simulink model "ANNModel"  (R2020a)
settings: Solver=VariableStepAuto  StartTime=0.0  StopTime=10.0  RelTol=1e-3
values from neighbouring files (symbols this model uses):
  dijastolniPritisak = str2num(get(handles.edit2,'string'))    [GUI.m]
  glukoza = str2num(get(handles.edit4,'string'))    [GUI.m]
  obimStruka = str2num(get(handles.edit1,'string'))    [GUI.m]
  sistolniPritisak = str2num(get(handles.edit3,'string'))    [GUI.m]
  trigliceridi = str2num(get(handles.edit5,'string'))    [GUI.m]
undefined symbols (not defined in the file or in its folder): hdlCartesian2PolarSetting
libraries: neural x255
(part 2 of 4)

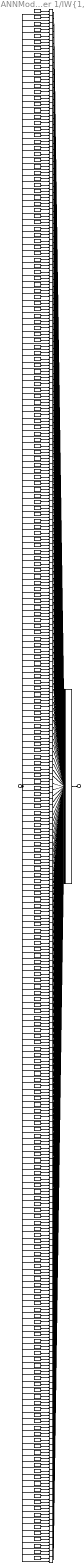
== system ANNModel/Function Fitting Neural Network/Layer 1/IW{1,1} ==
  "pd{1,1}" : Inport  PortDimensions=6
      mask Display: e = 0.06;c1 = [120 230 180]/255;c2 = ([120 230 180]+0)/(256+128);c3 = ([120 230 180]+128)/(256+128);patch([0 1 1 0],[0 0 1 1],c1);patch([0 1 1 1-e 1-e 0+e],[0 0 1 1-e 0+e 0+e],c2);patch([0 0 1 1-e 0+e 0+e],[0 1 1 1-e 1-e 0+e],c3);plot([0 1 1 0 0],[0 0 1 1 0]);
  "IW{1,1}(1,:)'" : Constant  Value=[0.287796190022346631831595686890068463981151580810546875;-1.9089648936896697062337580064195208251476287841796875;2.23832582693165793585876599536277353763580322265625;-1.4430056380304934204872324698953889310359954833984375;1.1609374416815703145999805201427079737186431884765625;-0.89544104034703086991697773555642925202846527099609375]
      mask Display: e = 0.06;c1 = [120 150 230]/255;c2 = ([120 150 230]+0)/383;c3 = ([120 150 230]+128)/383;patch([0 1 1 0],[0 0 1 1],c1);patch([0 1 1 1-e 1-e 0+e],[0 0 1 1-e 0+e 0+e],c2);patch([0 0 1 1-e 0+e 0+e],[0 1 1 1-e 1-e 0+e],c3);plot([0 1 1 0 0],[0 0 1 1 0]);disp('Weights');
  "IW{1,1}(10,:)'" : Constant  Value=[1.171278222760385734346755270962603390216827392578125;2.23653260652877516889702746993862092494964599609375;-0.01489189259019494011859752191639927332289516925811767578125;1.1450374400558178678011245210655033588409423828125;-1.8858407208954393041722141788341104984283447265625;-1.1545086890824993730575442896224558353424072265625]
      mask Display: e = 0.06;c1 = [120 150 230]/255;c2 = ([120 150 230]+0)/383;c3 = ([120 150 230]+128)/383;patch([0 1 1 0],[0 0 1 1],c1);patch([0 1 1 1-e 1-e 0+e],[0 0 1 1-e 0+e 0+e],c2);patch([0 0 1 1-e 0+e 0+e],[0 1 1 1-e 1-e 0+e],c3);plot([0 1 1 0 0],[0 0 1 1 0]);disp('Weights');
  "IW{1,1}(100,:)'" : Constant  Value=[1.663125101440811715036716122995130717754364013671875;-1.3324885457119133302938962515327148139476776123046875;1.40799126740946167757329021696932613849639892578125;-0.82146034869195483363313314839615486562252044677734375;-1.30446631893276876468235059292055666446685791015625;1.865641928271901672786725612240843474864959716796875]
      mask Display: e = 0.06;c1 = [120 150 230]/255;c2 = ([120 150 230]+0)/383;c3 = ([120 150 230]+128)/383;patch([0 1 1 0],[0 0 1 1],c1);patch([0 1 1 1-e 1-e 0+e],[0 0 1 1-e 0+e 0+e],c2);patch([0 0 1 1-e 0+e 0+e],[0 1 1 1-e 1-e 0+e],c3);plot([0 1 1 0 0],[0 0 1 1 0]);disp('Weights');
  "IW{1,1}(101,:)'" : Constant  Value=[1.0994399106034584701063749889726750552654266357421875;-1.94404946470914552492104121483862400054931640625;1.677632189897698022917893467820249497890472412109375;0.94695867514827247735098580960766412317752838134765625;-1.9872291711378233802776094307773746550083160400390625;0.461357489766259398766834465277497656643390655517578125]
      mask Display: e = 0.06;c1 = [120 150 230]/255;c2 = ([120 150 230]+0)/383;c3 = ([120 150 230]+128)/383;patch([0 1 1 0],[0 0 1 1],c1);patch([0 1 1 1-e 1-e 0+e],[0 0 1 1-e 0+e 0+e],c2);patch([0 0 1 1-e 0+e 0+e],[0 1 1 1-e 1-e 0+e],c3);plot([0 1 1 0 0],[0 0 1 1 0]);disp('Weights');
  "IW{1,1}(102,:)'" : Constant  Value=[-1.7449163202875137557157358969561755657196044921875;-0.9713941744906346986709877455723471939563751220703125;0.64768518707501609998899994025123305618762969970703125;1.7546407768395833048913345919572748243808746337890625;-2.00079378864895662815115429111756384372711181640625;-0.89837385215088028100893779992475174367427825927734375]
      mask Display: e = 0.06;c1 = [120 150 230]/255;c2 = ([120 150 230]+0)/383;c3 = ([120 150 230]+128)/383;patch([0 1 1 0],[0 0 1 1],c1);patch([0 1 1 1-e 1-e 0+e],[0 0 1 1-e 0+e 0+e],c2);patch([0 0 1 1-e 0+e 0+e],[0 1 1 1-e 1-e 0+e],c3);plot([0 1 1 0 0],[0 0 1 1 0]);disp('Weights');
  "IW{1,1}(103,:)'" : Constant  Value=[-1.8700045070212301112633213051594793796539306640625;1.1538376759129302939754779799841344356536865234375;1.3190542580864479393909505233750678598880767822265625;0.03391908880042536489352045236955746077001094818115234375;-1.42011272119921638790174256428144872188568115234375;-1.93961983755487921143867424689233303070068359375]
      mask Display: e = 0.06;c1 = [120 150 230]/255;c2 = ([120 150 230]+0)/383;c3 = ([120 150 230]+128)/383;patch([0 1 1 0],[0 0 1 1],c1);patch([0 1 1 1-e 1-e 0+e],[0 0 1 1-e 0+e 0+e],c2);patch([0 0 1 1-e 0+e 0+e],[0 1 1 1-e 1-e 0+e],c3);plot([0 1 1 0 0],[0 0 1 1 0]);disp('Weights');
  "IW{1,1}(104,:)'" : Constant  Value=[-1.9055149673777507235428174681146629154682159423828125;1.7368910868478895093147684747236780822277069091796875;-1.3775290622561680020652374878409318625926971435546875;-1.358849834002237688679315397166647017002105712890625;0.60619469881785248421834921828121878206729888916015625;-0.9743336437083087719912555257906205952167510986328125]
      mask Display: e = 0.06;c1 = [120 150 230]/255;c2 = ([120 150 230]+0)/383;c3 = ([120 150 230]+128)/383;patch([0 1 1 0],[0 0 1 1],c1);patch([0 1 1 1-e 1-e 0+e],[0 0 1 1-e 0+e 0+e],c2);patch([0 0 1 1-e 0+e 0+e],[0 1 1 1-e 1-e 0+e],c3);plot([0 1 1 0 0],[0 0 1 1 0]);disp('Weights');
  "IW{1,1}(105,:)'" : Constant  Value=[-1.2927935449414416080315959334257058799266815185546875;-2.876361513359648736098961308016441762447357177734375;0.144244721152042953971061933771125040948390960693359375;0.25663209727781233215893053056788630783557891845703125;0.58464584217745552141565212878049351274967193603515625;1.4202487725735595258669263785122893750667572021484375]
      mask Display: e = 0.06;c1 = [120 150 230]/255;c2 = ([120 150 230]+0)/383;c3 = ([120 150 230]+128)/383;patch([0 1 1 0],[0 0 1 1],c1);patch([0 1 1 1-e 1-e 0+e],[0 0 1 1-e 0+e 0+e],c2);patch([0 0 1 1-e 0+e 0+e],[0 1 1 1-e 1-e 0+e],c3);plot([0 1 1 0 0],[0 0 1 1 0]);disp('Weights');
  "IW{1,1}(106,:)'" : Constant  Value=[1.3715068673942329979809073847718536853790283203125;-1.8144972173688571626115617618779651820659637451171875;-1.659935553705334410068417128059081733226776123046875;-0.85473222772530255131329113282845355570316314697265625;1.8349805103916019266563353085075505077838897705078125;0.38149494665385663694223694619722664356231689453125]
      mask Display: e = 0.06;c1 = [120 150 230]/255;c2 = ([120 150 230]+0)/383;c3 = ([120 150 230]+128)/383;patch([0 1 1 0],[0 0 1 1],c1);patch([0 1 1 1-e 1-e 0+e],[0 0 1 1-e 0+e 0+e],c2);patch([0 0 1 1-e 0+e 0+e],[0 1 1 1-e 1-e 0+e],c3);plot([0 1 1 0 0],[0 0 1 1 0]);disp('Weights');
  "IW{1,1}(107,:)'" : Constant  Value=[-2.393727032684455746647245177882723510265350341796875;1.20553523596906675408035880536772310733795166015625;1.9170047359852304680316592566668987274169921875;-0.74935458790647413440666468886774964630603790283203125;0.827817899649488708746503107249736785888671875;0.400360585595414264492575284748454578220844268798828125]
      mask Display: e = 0.06;c1 = [120 150 230]/255;c2 = ([120 150 230]+0)/383;c3 = ([120 150 230]+128)/383;patch([0 1 1 0],[0 0 1 1],c1);patch([0 1 1 1-e 1-e 0+e],[0 0 1 1-e 0+e 0+e],c2);patch([0 0 1 1-e 0+e 0+e],[0 1 1 1-e 1-e 0+e],c3);plot([0 1 1 0 0],[0 0 1 1 0]);disp('Weights');
  "IW{1,1}(108,:)'" : Constant  Value=[0.58456128724172040644901926498278044164180755615234375;0.451576994767699135824301492903032340109348297119140625;-1.1295822098068881711441235893289558589458465576171875;-2.064741374551308350504541522241197526454925537109375;-0.330601885825315855438333301208331249654293060302734375;2.430200037822459080416592769324779510498046875]
      mask Display: e = 0.06;c1 = [120 150 230]/255;c2 = ([120 150 230]+0)/383;c3 = ([120 150 230]+128)/383;patch([0 1 1 0],[0 0 1 1],c1);patch([0 1 1 1-e 1-e 0+e],[0 0 1 1-e 0+e 0+e],c2);patch([0 0 1 1-e 0+e 0+e],[0 1 1 1-e 1-e 0+e],c3);plot([0 1 1 0 0],[0 0 1 1 0]);disp('Weights');
  "IW{1,1}(109,:)'" : Constant  Value=[2.180394306035542850707997786230407655239105224609375;-1.1778737761314694854064555329387076199054718017578125;2.11431337255463613900019481661729514598846435546875;1.1326449641214388908139198974822647869586944580078125;-0.67526687425978793033465308326412923634052276611328125;-0.07736857178589713612826272992606391198933124542236328125]
      mask Display: e = 0.06;c1 = [120 150 230]/255;c2 = ([120 150 230]+0)/383;c3 = ([120 150 230]+128)/383;patch([0 1 1 0],[0 0 1 1],c1);patch([0 1 1 1-e 1-e 0+e],[0 0 1 1-e 0+e 0+e],c2);patch([0 0 1 1-e 0+e 0+e],[0 1 1 1-e 1-e 0+e],c3);plot([0 1 1 0 0],[0 0 1 1 0]);disp('Weights');
  "IW{1,1}(11,:)'" : Constant  Value=[1.6315197961081737698663118862896226346492767333984375;-0.2131235197336888431696166890105814673006534576416015625;-0.815333650431852685613876019488088786602020263671875;2.37567903756769993606212665326893329620361328125;0.2414189732595966031425405162735842168331146240234375;-1.881982712422992864986781569314189255237579345703125]
      mask Display: e = 0.06;c1 = [120 150 230]/255;c2 = ([120 150 230]+0)/383;c3 = ([120 150 230]+128)/383;patch([0 1 1 0],[0 0 1 1],c1);patch([0 1 1 1-e 1-e 0+e],[0 0 1 1-e 0+e 0+e],c2);patch([0 0 1 1-e 0+e 0+e],[0 1 1 1-e 1-e 0+e],c3);plot([0 1 1 0 0],[0 0 1 1 0]);disp('Weights');
  "IW{1,1}(110,:)'" : Constant  Value=[1.871977750312087795947491031256504356861114501953125;1.9065529752603100899221999497967772185802459716796875;1.10235750480877481294328390504233539104461669921875;-0.12466250876593264196312560443402617238461971282958984375;-1.852760848460142550919727000291459262371063232421875;-0.83235765970877928499049858146463520824909210205078125]
      mask Display: e = 0.06;c1 = [120 150 230]/255;c2 = ([120 150 230]+0)/383;c3 = ([120 150 230]+128)/383;patch([0 1 1 0],[0 0 1 1],c1);patch([0 1 1 1-e 1-e 0+e],[0 0 1 1-e 0+e 0+e],c2);patch([0 0 1 1-e 0+e 0+e],[0 1 1 1-e 1-e 0+e],c3);plot([0 1 1 0 0],[0 0 1 1 0]);disp('Weights');
  "IW{1,1}(111,:)'" : Constant  Value=[2.715895301511082937651053725858218967914581298828125;-0.1845621160394123327908033616040484048426151275634765625;-1.1417582632765548300568525519338436424732208251953125;0.1105548504869580117571103983209468424320220947265625;-1.873172352911395943664274454931728541851043701171875;0.227437856943576932611250640547950752079486846923828125]
      mask Display: e = 0.06;c1 = [120 150 230]/255;c2 = ([120 150 230]+0)/383;c3 = ([120 150 230]+128)/383;patch([0 1 1 0],[0 0 1 1],c1);patch([0 1 1 1-e 1-e 0+e],[0 0 1 1-e 0+e 0+e],c2);patch([0 0 1 1-e 0+e 0+e],[0 1 1 1-e 1-e 0+e],c3);plot([0 1 1 0 0],[0 0 1 1 0]);disp('Weights');
  "IW{1,1}(112,:)'" : Constant  Value=[-2.865597023084187622288254715385846793651580810546875;0.55121427735391181901292156908311881124973297119140625;-1.3240199081592951557695414521731436252593994140625;1.03647974126135533623482842813245952129364013671875;-0.05899074146290349263122010370352654717862606048583984375;0.8046617095188033363939439368550665676593780517578125]
      mask Display: e = 0.06;c1 = [120 150 230]/255;c2 = ([120 150 230]+0)/383;c3 = ([120 150 230]+128)/383;patch([0 1 1 0],[0 0 1 1],c1);patch([0 1 1 1-e 1-e 0+e],[0 0 1 1-e 0+e 0+e],c2);patch([0 0 1 1-e 0+e 0+e],[0 1 1 1-e 1-e 0+e],c3);plot([0 1 1 0 0],[0 0 1 1 0]);disp('Weights');
  "IW{1,1}(113,:)'" : Constant  Value=[-0.310917571005290327423864482625504024326801300048828125;-0.785412215734894392227261050720699131488800048828125;-0.74616182881038906060666704433970153331756591796875;-2.010551802483051542225211960612796247005462646484375;-0.78039983614209218476531759733916260302066802978515625;-2.38104318153131000457278787507675588130950927734375]
      mask Display: e = 0.06;c1 = [120 150 230]/255;c2 = ([120 150 230]+0)/383;c3 = ([120 150 230]+128)/383;patch([0 1 1 0],[0 0 1 1],c1);patch([0 1 1 1-e 1-e 0+e],[0 0 1 1-e 0+e 0+e],c2);patch([0 0 1 1-e 0+e 0+e],[0 1 1 1-e 1-e 0+e],c3);plot([0 1 1 0 0],[0 0 1 1 0]);disp('Weights');
  "IW{1,1}(114,:)'" : Constant  Value=[-0.74016223365661082400634995792643167078495025634765625;-1.5122705125749271726220968048437498509883880615234375;-0.1761518912334952557952050256062648259103298187255859375;1.880329117756179169163033293443731963634490966796875;-1.4859694564245569115001899263006635010242462158203125;-1.9323614898229741765334210867877118289470672607421875]
      mask Display: e = 0.06;c1 = [120 150 230]/255;c2 = ([120 150 230]+0)/383;c3 = ([120 150 230]+128)/383;patch([0 1 1 0],[0 0 1 1],c1);patch([0 1 1 1-e 1-e 0+e],[0 0 1 1-e 0+e 0+e],c2);patch([0 0 1 1-e 0+e 0+e],[0 1 1 1-e 1-e 0+e],c3);plot([0 1 1 0 0],[0 0 1 1 0]);disp('Weights');
  "IW{1,1}(115,:)'" : Constant  Value=[-0.026530589428871730051096022862111567519605159759521484375;1.791368487953234112097788965911604464054107666015625;-0.038144839645352486556806326234436710365116596221923828125;1.3401104395405099012350547127425670623779296875;-1.646448745847335803915711949230171740055084228515625;-2.112684036522342267971907858736813068389892578125]
      mask Display: e = 0.06;c1 = [120 150 230]/255;c2 = ([120 150 230]+0)/383;c3 = ([120 150 230]+128)/383;patch([0 1 1 0],[0 0 1 1],c1);patch([0 1 1 1-e 1-e 0+e],[0 0 1 1-e 0+e 0+e],c2);patch([0 0 1 1-e 0+e 0+e],[0 1 1 1-e 1-e 0+e],c3);plot([0 1 1 0 0],[0 0 1 1 0]);disp('Weights');
  "IW{1,1}(116,:)'" : Constant  Value=[1.5812661283949827062400572685874067246913909912109375;1.767995003883346072370841284282505512237548828125;-0.346389538115326522937920117328758351504802703857421875;0.431948010021581618733677032651030458509922027587890625;-1.8555401924967716009717833003378473222255706787109375;-1.704494922192528516546872197068296372890472412109375]
      mask Display: e = 0.06;c1 = [120 150 230]/255;c2 = ([120 150 230]+0)/383;c3 = ([120 150 230]+128)/383;patch([0 1 1 0],[0 0 1 1],c1);patch([0 1 1 1-e 1-e 0+e],[0 0 1 1-e 0+e 0+e],c2);patch([0 0 1 1-e 0+e 0+e],[0 1 1 1-e 1-e 0+e],c3);plot([0 1 1 0 0],[0 0 1 1 0]);disp('Weights');
  "IW{1,1}(117,:)'" : Constant  Value=[-1.2368412784026714401619528871378861367702484130859375;2.249261562349092802293171189376153051853179931640625;0.69995883312456508296151014292263425886631011962890625;0.089521939729461597057280641820398159325122833251953125;1.177139767436751416340712239616550505161285400390625;-1.871593531701182921977988371509127318859100341796875]
      mask Display: e = 0.06;c1 = [120 150 230]/255;c2 = ([120 150 230]+0)/383;c3 = ([120 150 230]+128)/383;patch([0 1 1 0],[0 0 1 1],c1);patch([0 1 1 1-e 1-e 0+e],[0 0 1 1-e 0+e 0+e],c2);patch([0 0 1 1-e 0+e 0+e],[0 1 1 1-e 1-e 0+e],c3);plot([0 1 1 0 0],[0 0 1 1 0]);disp('Weights');
  "IW{1,1}(118,:)'" : Constant  Value=[0.60304962449617349751207484587212093174457550048828125;-1.124505931275801007274139919900335371494293212890625;-2.198952551738090566146865967311896383762359619140625;-1.0802931006421128135031040073954500257968902587890625;-0.89556215647179382433051841871929354965686798095703125;1.944692625398790841728668965515680611133575439453125]
      mask Display: e = 0.06;c1 = [120 150 230]/255;c2 = ([120 150 230]+0)/383;c3 = ([120 150 230]+128)/383;patch([0 1 1 0],[0 0 1 1],c1);patch([0 1 1 1-e 1-e 0+e],[0 0 1 1-e 0+e 0+e],c2);patch([0 0 1 1-e 0+e 0+e],[0 1 1 1-e 1-e 0+e],c3);plot([0 1 1 0 0],[0 0 1 1 0]);disp('Weights');
  "IW{1,1}(119,:)'" : Constant  Value=[1.482736380110039942081812114338390529155731201171875;-0.6897419204355188515620511680026538670063018798828125;-0.7221616959874612717840136610902845859527587890625;1.878595439276721013044380015344358980655670166015625;1.0859477348788020290015765567659400403499603271484375;-2.0840921036468404992092473548837006092071533203125]
      mask Display: e = 0.06;c1 = [120 150 230]/255;c2 = ([120 150 230]+0)/383;c3 = ([120 150 230]+128)/383;patch([0 1 1 0],[0 0 1 1],c1);patch([0 1 1 1-e 1-e 0+e],[0 0 1 1-e 0+e 0+e],c2);patch([0 0 1 1-e 0+e 0+e],[0 1 1 1-e 1-e 0+e],c3);plot([0 1 1 0 0],[0 0 1 1 0]);disp('Weights');
  "IW{1,1}(12,:)'" : Constant  Value=[1.5455546652351539460568119466188363730907440185546875;-1.5484718191601032355464440115611068904399871826171875;1.7087711909293610279547692698542959988117218017578125;1.785864571327177241499839510652236640453338623046875;1.4157761391038483633764144542510621249675750732421875;-1.5651679421094624178323329033446498215198516845703125]
      mask Display: e = 0.06;c1 = [120 150 230]/255;c2 = ([120 150 230]+0)/383;c3 = ([120 150 230]+128)/383;patch([0 1 1 0],[0 0 1 1],c1);patch([0 1 1 1-e 1-e 0+e],[0 0 1 1-e 0+e 0+e],c2);patch([0 0 1 1-e 0+e 0+e],[0 1 1 1-e 1-e 0+e],c3);plot([0 1 1 0 0],[0 0 1 1 0]);disp('Weights');
  "IW{1,1}(120,:)'" : Constant  Value=[1.288138171530183395674384883022867143154144287109375;1.7591734283443953845704754712642170488834381103515625;-2.546961424497379056219870108179748058319091796875;0.26152048374034009281530188673059456050395965576171875;-0.75234596311726098516459160236991010606288909912109375;-0.396041123684448159725235427686129696667194366455078125]
      mask Display: e = 0.06;c1 = [120 150 230]/255;c2 = ([120 150 230]+0)/383;c3 = ([120 150 230]+128)/383;patch([0 1 1 0],[0 0 1 1],c1);patch([0 1 1 1-e 1-e 0+e],[0 0 1 1-e 0+e 0+e],c2);patch([0 0 1 1-e 0+e 0+e],[0 1 1 1-e 1-e 0+e],c3);plot([0 1 1 0 0],[0 0 1 1 0]);disp('Weights');
  "IW{1,1}(121,:)'" : Constant  Value=[1.6789379176582592823052664243732579052448272705078125;-2.06756931519347464387692525633610785007476806640625;-0.83431558709326869571754059506929479539394378662109375;-0.11764986868161116106978880679889698512852191925048828125;-0.741921904057246894836907813441939651966094970703125;1.7037612455942536815456378462840802967548370361328125]
      mask Display: e = 0.06;c1 = [120 150 230]/255;c2 = ([120 150 230]+0)/383;c3 = ([120 150 230]+128)/383;patch([0 1 1 0],[0 0 1 1],c1);patch([0 1 1 1-e 1-e 0+e],[0 0 1 1-e 0+e 0+e],c2);patch([0 0 1 1-e 0+e 0+e],[0 1 1 1-e 1-e 0+e],c3);plot([0 1 1 0 0],[0 0 1 1 0]);disp('Weights');
  "IW{1,1}(122,:)'" : Constant  Value=[-2.597069193765010997054787367233075201511383056640625;0.443010847045192390769585699672461487352848052978515625;-0.916897332638182849251506922882981598377227783203125;1.6149206099324933116889724260545335710048675537109375;-1.4291647808392660135012874889071099460124969482421875;-0.011755427704555405921116317813357454724609851837158203125]
      mask Display: e = 0.06;c1 = [120 150 230]/255;c2 = ([120 150 230]+0)/383;c3 = ([120 150 230]+128)/383;patch([0 1 1 0],[0 0 1 1],c1);patch([0 1 1 1-e 1-e 0+e],[0 0 1 1-e 0+e 0+e],c2);patch([0 0 1 1-e 0+e 0+e],[0 1 1 1-e 1-e 0+e],c3);plot([0 1 1 0 0],[0 0 1 1 0]);disp('Weights');
  "IW{1,1}(123,:)'" : Constant  Value=[1.82950962756301027667404923704452812671661376953125;-0.766808582879284994504587302799336612224578857421875;-1.96057973625015602436860717716626822948455810546875;1.0438555136353444563468428896158002316951751708984375;-0.937696667328782762496075520175509154796600341796875;-1.5015461343558171858347805027733556926250457763671875]
      mask Display: e = 0.06;c1 = [120 150 230]/255;c2 = ([120 150 230]+0)/383;c3 = ([120 150 230]+128)/383;patch([0 1 1 0],[0 0 1 1],c1);patch([0 1 1 1-e 1-e 0+e],[0 0 1 1-e 0+e 0+e],c2);patch([0 0 1 1-e 0+e 0+e],[0 1 1 1-e 1-e 0+e],c3);plot([0 1 1 0 0],[0 0 1 1 0]);disp('Weights');
  "IW{1,1}(124,:)'" : Constant  Value=[-1.717308648500118994917329473537392914295196533203125;-0.1143933240111000559924292474534013308584690093994140625;0.70796833666341374424746391014195978641510009765625;1.6833517489322911142579641818883828818798065185546875;-1.6455079596563706445522257126867771148681640625;1.8053204278844316998942076679668389260768890380859375]
      mask Display: e = 0.06;c1 = [120 150 230]/255;c2 = ([120 150 230]+0)/383;c3 = ([120 150 230]+128)/383;patch([0 1 1 0],[0 0 1 1],c1);patch([0 1 1 1-e 1-e 0+e],[0 0 1 1-e 0+e 0+e],c2);patch([0 0 1 1-e 0+e 0+e],[0 1 1 1-e 1-e 0+e],c3);plot([0 1 1 0 0],[0 0 1 1 0]);disp('Weights');
  "IW{1,1}(125,:)'" : Constant  Value=[1.2768026276094157633878012347850017249584197998046875;-1.4743738311023104614605472306720912456512451171875;0.689266690328770526008383967564441263675689697265625;0.449442201861272982998940506149665452539920806884765625;1.553334665702312822332942232606001198291778564453125;2.238972463563259740482180859544314444065093994140625]
      mask Display: e = 0.06;c1 = [120 150 230]/255;c2 = ([120 150 230]+0)/383;c3 = ([120 150 230]+128)/383;patch([0 1 1 0],[0 0 1 1],c1);patch([0 1 1 1-e 1-e 0+e],[0 0 1 1-e 0+e 0+e],c2);patch([0 0 1 1-e 0+e 0+e],[0 1 1 1-e 1-e 0+e],c3);plot([0 1 1 0 0],[0 0 1 1 0]);disp('Weights');
  "IW{1,1}(126,:)'" : Constant  Value=[1.185869669339465470869754426530562341213226318359375;-1.8183989232825459314568661284283734858036041259765625;1.4622955843601552761157336135511286556720733642578125;-1.31858677302676507991918697371147572994232177734375;-1.3866742775623348560287695363513194024562835693359375;0.8449734256742991167499212679103948175907135009765625]
      mask Display: e = 0.06;c1 = [120 150 230]/255;c2 = ([120 150 230]+0)/383;c3 = ([120 150 230]+128)/383;patch([0 1 1 0],[0 0 1 1],c1);patch([0 1 1 1-e 1-e 0+e],[0 0 1 1-e 0+e 0+e],c2);patch([0 0 1 1-e 0+e 0+e],[0 1 1 1-e 1-e 0+e],c3);plot([0 1 1 0 0],[0 0 1 1 0]);disp('Weights');
  "IW{1,1}(127,:)'" : Constant  Value=[-1.5208700661502623230347808203077875077724456787109375;0.36918303584951883689058149684569798409938812255859375;-0.67113679415553428864171792156412266194820404052734375;-1.609631995417881711318841553293168544769287109375;-1.9015268710997628165415562762063927948474884033203125;-1.85020841591162987782581694773398339748382568359375]
      mask Display: e = 0.06;c1 = [120 150 230]/255;c2 = ([120 150 230]+0)/383;c3 = ([120 150 230]+128)/383;patch([0 1 1 0],[0 0 1 1],c1);patch([0 1 1 1-e 1-e 0+e],[0 0 1 1-e 0+e 0+e],c2);patch([0 0 1 1-e 0+e 0+e],[0 1 1 1-e 1-e 0+e],c3);plot([0 1 1 0 0],[0 0 1 1 0]);disp('Weights');
  "IW{1,1}(128,:)'" : Constant  Value=[2.244153766149360240689247802947647869586944580078125;-0.285950788072386996585549923111102543771266937255859375;0.75772497186099785349000512724160216748714447021484375;-1.8382734286454243122221896555856801569461822509765625;-1.05364333862193060298295677057467401027679443359375;-1.5863157094262325674804969821707345545291900634765625]
      mask Display: e = 0.06;c1 = [120 150 230]/255;c2 = ([120 150 230]+0)/383;c3 = ([120 150 230]+128)/383;patch([0 1 1 0],[0 0 1 1],c1);patch([0 1 1 1-e 1-e 0+e],[0 0 1 1-e 0+e 0+e],c2);patch([0 0 1 1-e 0+e 0+e],[0 1 1 1-e 1-e 0+e],c3);plot([0 1 1 0 0],[0 0 1 1 0]);disp('Weights');
  "IW{1,1}(129,:)'" : Constant  Value=[-1.3295196024708582083206920287921093404293060302734375;-0.98565154486492290164534324503620155155658721923828125;0.60676632133203156627132557332515716552734375;-1.672370422375341281195915144053287804126739501953125;1.6587910150941505005306453313096426427364349365234375;-1.8893294430765006364225655488553456962108612060546875]
      mask Display: e = 0.06;c1 = [120 150 230]/255;c2 = ([120 150 230]+0)/383;c3 = ([120 150 230]+128)/383;patch([0 1 1 0],[0 0 1 1],c1);patch([0 1 1 1-e 1-e 0+e],[0 0 1 1-e 0+e 0+e],c2);patch([0 0 1 1-e 0+e 0+e],[0 1 1 1-e 1-e 0+e],c3);plot([0 1 1 0 0],[0 0 1 1 0]);disp('Weights');
  "IW{1,1}(13,:)'" : Constant  Value=[0.81921892677472640809099857506225816905498504638671875;1.568457929113170390422737909830175340175628662109375;2.04499941443174382271763533935882151126861572265625;-1.5514905638126545994737170985899865627288818359375;-1.529102764073087872276346388389356434345245361328125;-0.92744381079182913740766025512129999697208404541015625]
      mask Display: e = 0.06;c1 = [120 150 230]/255;c2 = ([120 150 230]+0)/383;c3 = ([120 150 230]+128)/383;patch([0 1 1 0],[0 0 1 1],c1);patch([0 1 1 1-e 1-e 0+e],[0 0 1 1-e 0+e 0+e],c2);patch([0 0 1 1-e 0+e 0+e],[0 1 1 1-e 1-e 0+e],c3);plot([0 1 1 0 0],[0 0 1 1 0]);disp('Weights');
  "IW{1,1}(130,:)'" : Constant  Value=[2.408864728766730411990693028201349079608917236328125;-0.423623329771535550580807694132090546190738677978515625;-1.1495083404988843955862876100582070648670196533203125;-0.58093209613445784267327098859823308885097503662109375;-2.0011779217500862415590745513327419757843017578125;-0.2364424998863863536247009733415325172245502471923828125]
      mask Display: e = 0.06;c1 = [120 150 230]/255;c2 = ([120 150 230]+0)/383;c3 = ([120 150 230]+128)/383;patch([0 1 1 0],[0 0 1 1],c1);patch([0 1 1 1-e 1-e 0+e],[0 0 1 1-e 0+e 0+e],c2);patch([0 0 1 1-e 0+e 0+e],[0 1 1 1-e 1-e 0+e],c3);plot([0 1 1 0 0],[0 0 1 1 0]);disp('Weights');
  "IW{1,1}(131,:)'" : Constant  Value=[-1.5353181139611884464812874284689314663410186767578125;-0.229523342731099033731112513123662211000919342041015625;-1.042883638094376674843033470096997916698455810546875;1.0970742301310634214672745656571350991725921630859375;-0.78281070984578438043399728485383093357086181640625;2.49132644022129046135205499012954533100128173828125]
      mask Display: e = 0.06;c1 = [120 150 230]/255;c2 = ([120 150 230]+0)/383;c3 = ([120 150 230]+128)/383;patch([0 1 1 0],[0 0 1 1],c1);patch([0 1 1 1-e 1-e 0+e],[0 0 1 1-e 0+e 0+e],c2);patch([0 0 1 1-e 0+e 0+e],[0 1 1 1-e 1-e 0+e],c3);plot([0 1 1 0 0],[0 0 1 1 0]);disp('Weights');
  "IW{1,1}(132,:)'" : Constant  Value=[1.4011749553231862552848951963824220001697540283203125;2.774769041384399503868962710839696228504180908203125;1.32885152716597421118649435811676084995269775390625;-0.770037401136249854971538297832012176513671875;0.305191395473012716532679178271791897714138031005859375;0.499106448584099637866273724284837953746318817138671875]
      mask Display: e = 0.06;c1 = [120 150 230]/255;c2 = ([120 150 230]+0)/383;c3 = ([120 150 230]+128)/383;patch([0 1 1 0],[0 0 1 1],c1);patch([0 1 1 1-e 1-e 0+e],[0 0 1 1-e 0+e 0+e],c2);patch([0 0 1 1-e 0+e 0+e],[0 1 1 1-e 1-e 0+e],c3);plot([0 1 1 0 0],[0 0 1 1 0]);disp('Weights');
  "IW{1,1}(133,:)'" : Constant  Value=[0.410349731679175822041116816762951202690601348876953125;-0.6737885367440743511480150118586607277393341064453125;-2.439852619469064176627171036670915782451629638671875;-2.287856232914155629742936071124859154224395751953125;0.0761743555694443796877379782017669640481472015380859375;-0.45265290741523955819758384677697904407978057861328125]
      mask Display: e = 0.06;c1 = [120 150 230]/255;c2 = ([120 150 230]+0)/383;c3 = ([120 150 230]+128)/383;patch([0 1 1 0],[0 0 1 1],c1);patch([0 1 1 1-e 1-e 0+e],[0 0 1 1-e 0+e 0+e],c2);patch([0 0 1 1-e 0+e 0+e],[0 1 1 1-e 1-e 0+e],c3);plot([0 1 1 0 0],[0 0 1 1 0]);disp('Weights');
  "IW{1,1}(134,:)'" : Constant  Value=[-1.5396312738240405249001696574850939214229583740234375;1.19216090099692184622881541145034134387969970703125;1.68856762666094795122262439690530300140380859375;-1.740367974127239758530549806891940534114837646484375;1.3443872921924400198889770763344131410121917724609375;0.0064487849477914589713112292201913078315556049346923828125]
      mask Display: e = 0.06;c1 = [120 150 230]/255;c2 = ([120 150 230]+0)/383;c3 = ([120 150 230]+128)/383;patch([0 1 1 0],[0 0 1 1],c1);patch([0 1 1 1-e 1-e 0+e],[0 0 1 1-e 0+e 0+e],c2);patch([0 0 1 1-e 0+e 0+e],[0 1 1 1-e 1-e 0+e],c3);plot([0 1 1 0 0],[0 0 1 1 0]);disp('Weights');
  "IW{1,1}(135,:)'" : Constant  Value=[-1.2882945544971631246511378776631318032741546630859375;-0.93848015616414215411822397072683088481426239013671875;0.5476472316385156968721048542647622525691986083984375;0.677561346607494119353987116483040153980255126953125;-2.377698237015096083268872462213039398193359375;-1.384561142424645563409058013348840177059173583984375]
      mask Display: e = 0.06;c1 = [120 150 230]/255;c2 = ([120 150 230]+0)/383;c3 = ([120 150 230]+128)/383;patch([0 1 1 0],[0 0 1 1],c1);patch([0 1 1 1-e 1-e 0+e],[0 0 1 1-e 0+e 0+e],c2);patch([0 0 1 1-e 0+e 0+e],[0 1 1 1-e 1-e 0+e],c3);plot([0 1 1 0 0],[0 0 1 1 0]);disp('Weights');
  "IW{1,1}(136,:)'" : Constant  Value=[-1.72156266778102118308879653341136872768402099609375;-1.068743812235457557591189470258541405200958251953125;-1.5335392213944454287144480986171402037143707275390625;1.044227060616664370940043227165006101131439208984375;1.5141058820249586602812996716238558292388916015625;1.2801488802897711405393010863917879760265350341796875]
      mask Display: e = 0.06;c1 = [120 150 230]/255;c2 = ([120 150 230]+0)/383;c3 = ([120 150 230]+128)/383;patch([0 1 1 0],[0 0 1 1],c1);patch([0 1 1 1-e 1-e 0+e],[0 0 1 1-e 0+e 0+e],c2);patch([0 0 1 1-e 0+e 0+e],[0 1 1 1-e 1-e 0+e],c3);plot([0 1 1 0 0],[0 0 1 1 0]);disp('Weights');
  "IW{1,1}(137,:)'" : Constant  Value=[1.7212827915591935035166670786566101014614105224609375;-1.1027546621857313713377379826852120459079742431640625;1.5388616316426695362906684749759733676910400390625;-1.7112085547187092515741824172437191009521484375;1.6534100705921914720164522805134765803813934326171875;-0.57240716144628311923270302941091358661651611328125]
      mask Display: e = 0.06;c1 = [120 150 230]/255;c2 = ([120 150 230]+0)/383;c3 = ([120 150 230]+128)/383;patch([0 1 1 0],[0 0 1 1],c1);patch([0 1 1 1-e 1-e 0+e],[0 0 1 1-e 0+e 0+e],c2);patch([0 0 1 1-e 0+e 0+e],[0 1 1 1-e 1-e 0+e],c3);plot([0 1 1 0 0],[0 0 1 1 0]);disp('Weights');
  "IW{1,1}(138,:)'" : Constant  Value=[0.3139608338656565411639576268498785793781280517578125;1.1973681996248617398492797292419709265232086181640625;-0.2029654646614268143078874118145904503762722015380859375;-1.6199100315220091861334594796062447130680084228515625;2.438351611880173575030994470580480992794036865234375;1.3652432569773143011815363934147171676158905029296875]
      mask Display: e = 0.06;c1 = [120 150 230]/255;c2 = ([120 150 230]+0)/383;c3 = ([120 150 230]+128)/383;patch([0 1 1 0],[0 0 1 1],c1);patch([0 1 1 1-e 1-e 0+e],[0 0 1 1-e 0+e 0+e],c2);patch([0 0 1 1-e 0+e 0+e],[0 1 1 1-e 1-e 0+e],c3);plot([0 1 1 0 0],[0 0 1 1 0]);disp('Weights');
  "IW{1,1}(139,:)'" : Constant  Value=[1.997301106317598051731465602642856538295745849609375;0.59780683624300079426205911659053526818752288818359375;2.056219592138236240685955635854043066501617431640625;-0.161815986942669021164675768886809237301349639892578125;-1.6570841122033799219792626900016330182552337646484375;-0.72123634029240724085951796951121650636196136474609375]
      mask Display: e = 0.06;c1 = [120 150 230]/255;c2 = ([120 150 230]+0)/383;c3 = ([120 150 230]+128)/383;patch([0 1 1 0],[0 0 1 1],c1);patch([0 1 1 1-e 1-e 0+e],[0 0 1 1-e 0+e 0+e],c2);patch([0 0 1 1-e 0+e 0+e],[0 1 1 1-e 1-e 0+e],c3);plot([0 1 1 0 0],[0 0 1 1 0]);disp('Weights');
  "IW{1,1}(14,:)'" : Constant  Value=[1.700544810453186617138499059365130960941314697265625;-2.511617508302337764547473852871917188167572021484375;0.135653647038074975927912646511686034500598907470703125;0.6767325351837081282013741656555794179439544677734375;-0.715991092657897620910034675034694373607635498046875;-1.396603283186203636745403855456970632076263427734375]
      mask Display: e = 0.06;c1 = [120 150 230]/255;c2 = ([120 150 230]+0)/383;c3 = ([120 150 230]+128)/383;patch([0 1 1 0],[0 0 1 1],c1);patch([0 1 1 1-e 1-e 0+e],[0 0 1 1-e 0+e 0+e],c2);patch([0 0 1 1-e 0+e 0+e],[0 1 1 1-e 1-e 0+e],c3);plot([0 1 1 0 0],[0 0 1 1 0]);disp('Weights');
  "IW{1,1}(140,:)'" : Constant  Value=[-1.086234892153952191762300572008825838565826416015625;1.765273255568697408079970045946538448333740234375;1.81656433443234721636372341890819370746612548828125;-0.8113781534170192433208512738929130136966705322265625;-1.4608225218397736799857966616400517523288726806640625;-1.3105318241304566573290912856464274227619171142578125]
      mask Display: e = 0.06;c1 = [120 150 230]/255;c2 = ([120 150 230]+0)/383;c3 = ([120 150 230]+128)/383;patch([0 1 1 0],[0 0 1 1],c1);patch([0 1 1 1-e 1-e 0+e],[0 0 1 1-e 0+e 0+e],c2);patch([0 0 1 1-e 0+e 0+e],[0 1 1 1-e 1-e 0+e],c3);plot([0 1 1 0 0],[0 0 1 1 0]);disp('Weights');
  "IW{1,1}(141,:)'" : Constant  Value=[0.70837803361070406094057716472889296710491180419921875;2.34832250059937397423936999985016882419586181640625;-1.05225138900724335400127529283054172992706298828125;0.450613094512413658865312982015893794596195220947265625;-0.7854690921748159748716489048092626035213470458984375;-1.9256366113215925839341480241273529827594757080078125]
      mask Display: e = 0.06;c1 = [120 150 230]/255;c2 = ([120 150 230]+0)/383;c3 = ([120 150 230]+128)/383;patch([0 1 1 0],[0 0 1 1],c1);patch([0 1 1 1-e 1-e 0+e],[0 0 1 1-e 0+e 0+e],c2);patch([0 0 1 1-e 0+e 0+e],[0 1 1 1-e 1-e 0+e],c3);plot([0 1 1 0 0],[0 0 1 1 0]);disp('Weights');
  "IW{1,1}(142,:)'" : Constant  Value=[1.86843860515786897025236612535081803798675537109375;1.6787359647101707249561286516836844384670257568359375;0.202945741843797267112137205913313664495944976806640625;1.7110247230668964579791690994170494377613067626953125;-0.2013491983710975208321514173803734593093395233154296875;1.425668001528340500527747281012125313282012939453125]
      mask Display: e = 0.06;c1 = [120 150 230]/255;c2 = ([120 150 230]+0)/383;c3 = ([120 150 230]+128)/383;patch([0 1 1 0],[0 0 1 1],c1);patch([0 1 1 1-e 1-e 0+e],[0 0 1 1-e 0+e 0+e],c2);patch([0 0 1 1-e 0+e 0+e],[0 1 1 1-e 1-e 0+e],c3);plot([0 1 1 0 0],[0 0 1 1 0]);disp('Weights');
  "IW{1,1}(143,:)'" : Constant  Value=[-0.60008071271782659206195376100367866456508636474609375;0.82076341229811899946611220002523623406887054443359375;-2.6729897971959903912875233800150454044342041015625;0.783311403201848666100204354734160006046295166015625;0.52599991018321434754767551567056216299533843994140625;1.781241346979083317592085222713649272918701171875]
      mask Display: e = 0.06;c1 = [120 150 230]/255;c2 = ([120 150 230]+0)/383;c3 = ([120 150 230]+128)/383;patch([0 1 1 0],[0 0 1 1],c1);patch([0 1 1 1-e 1-e 0+e],[0 0 1 1-e 0+e 0+e],c2);patch([0 0 1 1-e 0+e 0+e],[0 1 1 1-e 1-e 0+e],c3);plot([0 1 1 0 0],[0 0 1 1 0]);disp('Weights');
  "IW{1,1}(144,:)'" : Constant  Value=[1.509612652085633666132480357191525399684906005859375;1.557821267941999821005083504132926464080810546875;-1.424267368498784325225869906716980040073394775390625;1.745698658741959174989233360975049436092376708984375;1.462230922523412690594568630331195890903472900390625;-0.5831118049386792012711566712823696434497833251953125]
      mask Display: e = 0.06;c1 = [120 150 230]/255;c2 = ([120 150 230]+0)/383;c3 = ([120 150 230]+128)/383;patch([0 1 1 0],[0 0 1 1],c1);patch([0 1 1 1-e 1-e 0+e],[0 0 1 1-e 0+e 0+e],c2);patch([0 0 1 1-e 0+e 0+e],[0 1 1 1-e 1-e 0+e],c3);plot([0 1 1 0 0],[0 0 1 1 0]);disp('Weights');
  "IW{1,1}(145,:)'" : Constant  Value=[-1.7732167623160222102995930981705896556377410888671875;0.15002483172881075912385995252407155930995941162109375;-0.886374102116904705184197155176661908626556396484375;0.97189791592051621993419985301443375647068023681640625;1.5499905337623498535748467475059442222118377685546875;-2.2422384466302052175024073221720755100250244140625]
      mask Display: e = 0.06;c1 = [120 150 230]/255;c2 = ([120 150 230]+0)/383;c3 = ([120 150 230]+128)/383;patch([0 1 1 0],[0 0 1 1],c1);patch([0 1 1 1-e 1-e 0+e],[0 0 1 1-e 0+e 0+e],c2);patch([0 0 1 1-e 0+e 0+e],[0 1 1 1-e 1-e 0+e],c3);plot([0 1 1 0 0],[0 0 1 1 0]);disp('Weights');
  "IW{1,1}(146,:)'" : Constant  Value=[-1.61902336602567498147209335002116858959197998046875;-0.28818642435812147351015255480888299643993377685546875;1.331311491473435193455543412710539996623992919921875;0.113949860816193793144890378243871964514255523681640625;1.0247089261697797102357299081631936132907867431640625;-2.600254605954875675166704240837134420871734619140625]
      mask Display: e = 0.06;c1 = [120 150 230]/255;c2 = ([120 150 230]+0)/383;c3 = ([120 150 230]+128)/383;patch([0 1 1 0],[0 0 1 1],c1);patch([0 1 1 1-e 1-e 0+e],[0 0 1 1-e 0+e 0+e],c2);patch([0 0 1 1-e 0+e 0+e],[0 1 1 1-e 1-e 0+e],c3);plot([0 1 1 0 0],[0 0 1 1 0]);disp('Weights');
  "IW{1,1}(147,:)'" : Constant  Value=[-0.73015481589031583364857169726747088134288787841796875;-1.26795890093057739278492590528912842273712158203125;-0.946679033493526222997616059728898108005523681640625;2.3140663930235714218497378169558942317962646484375;-0.132591643545464876741135640259017236530780792236328125;1.97381713218176191304564781603403389453887939453125]
      mask Display: e = 0.06;c1 = [120 150 230]/255;c2 = ([120 150 230]+0)/383;c3 = ([120 150 230]+128)/383;patch([0 1 1 0],[0 0 1 1],c1);patch([0 1 1 1-e 1-e 0+e],[0 0 1 1-e 0+e 0+e],c2);patch([0 0 1 1-e 0+e 0+e],[0 1 1 1-e 1-e 0+e],c3);plot([0 1 1 0 0],[0 0 1 1 0]);disp('Weights');
  "IW{1,1}(148,:)'" : Constant  Value=[-1.46359104229331382640566516784019768238067626953125;1.320149975572655787203757427050732076168060302734375;0.2092767184015128234531033513121656142175197601318359375;-2.408576276263271864763737539760768413543701171875;-0.66705784676068635707935072787222452461719512939453125;-1.44098196375615383857393680955283343791961669921875]
      mask Display: e = 0.06;c1 = [120 150 230]/255;c2 = ([120 150 230]+0)/383;c3 = ([120 150 230]+128)/383;patch([0 1 1 0],[0 0 1 1],c1);patch([0 1 1 1-e 1-e 0+e],[0 0 1 1-e 0+e 0+e],c2);patch([0 0 1 1-e 0+e 0+e],[0 1 1 1-e 1-e 0+e],c3);plot([0 1 1 0 0],[0 0 1 1 0]);disp('Weights');
  "IW{1,1}(149,:)'" : Constant  Value=[-1.326508557398286658468578025349415838718414306640625;0.63039628744379161418009971384890377521514892578125;-0.48969420370395499997329125108080916106700897216796875;-2.7051583542840429430498261353932321071624755859375;0.383557547686325495117642958575743250548839569091796875;1.49224283392324519326166409882716834545135498046875]
      mask Display: e = 0.06;c1 = [120 150 230]/255;c2 = ([120 150 230]+0)/383;c3 = ([120 150 230]+128)/383;patch([0 1 1 0],[0 0 1 1],c1);patch([0 1 1 1-e 1-e 0+e],[0 0 1 1-e 0+e 0+e],c2);patch([0 0 1 1-e 0+e 0+e],[0 1 1 1-e 1-e 0+e],c3);plot([0 1 1 0 0],[0 0 1 1 0]);disp('Weights');
  "IW{1,1}(15,:)'" : Constant  Value=[-0.7990390817567625258988073255750350654125213623046875;-1.3787527530744281278884955099783837795257568359375;0.265506645175145161719143516165786422789096832275390625;1.334295142977879766732485222746618092060089111328125;-2.297705824550424491548028527176938951015472412109375;-1.548002609162630438532914922689087688922882080078125]
      mask Display: e = 0.06;c1 = [120 150 230]/255;c2 = ([120 150 230]+0)/383;c3 = ([120 150 230]+128)/383;patch([0 1 1 0],[0 0 1 1],c1);patch([0 1 1 1-e 1-e 0+e],[0 0 1 1-e 0+e 0+e],c2);patch([0 0 1 1-e 0+e 0+e],[0 1 1 1-e 1-e 0+e],c3);plot([0 1 1 0 0],[0 0 1 1 0]);disp('Weights');
  "IW{1,1}(150,:)'" : Constant  Value=[1.9835699277077678548408812275738455355167388916015625;-1.9443006282396269046586212425609119236469268798828125;1.0470610633865689020893796623568050563335418701171875;1.764942625596600311865813637268729507923126220703125;0.29732042957043436359754196018911898136138916015625;-0.04224876694125954956771096249212860129773616790771484375]
      mask Display: e = 0.06;c1 = [120 150 230]/255;c2 = ([120 150 230]+0)/383;c3 = ([120 150 230]+128)/383;patch([0 1 1 0],[0 0 1 1],c1);patch([0 1 1 1-e 1-e 0+e],[0 0 1 1-e 0+e 0+e],c2);patch([0 0 1 1-e 0+e 0+e],[0 1 1 1-e 1-e 0+e],c3);plot([0 1 1 0 0],[0 0 1 1 0]);disp('Weights');
  "IW{1,1}(151,:)'" : Constant  Value=[0.54864589249590578479143232470960356295108795166015625;0.7186186069536255605072483376716263592243194580078125;2.132898076963197109279235519352369010448455810546875;-0.41957251800809591824048538910574279725551605224609375;-2.058481140764126138265055487863719463348388671875;1.5646670365955130943547146671335212886333465576171875]
      mask Display: e = 0.06;c1 = [120 150 230]/255;c2 = ([120 150 230]+0)/383;c3 = ([120 150 230]+128)/383;patch([0 1 1 0],[0 0 1 1],c1);patch([0 1 1 1-e 1-e 0+e],[0 0 1 1-e 0+e 0+e],c2);patch([0 0 1 1-e 0+e 0+e],[0 1 1 1-e 1-e 0+e],c3);plot([0 1 1 0 0],[0 0 1 1 0]);disp('Weights');
  "IW{1,1}(152,:)'" : Constant  Value=[0.53330210891901097536305087487562559545040130615234375;2.317341007173086442350040670135058462619781494140625;-0.2948378446817991882511478252126835286617279052734375;1.14459374416777759364549638121388852596282958984375;1.701722907085264413495906410389579832553863525390625;-1.1939601185085486623194128696923144161701202392578125]
      mask Display: e = 0.06;c1 = [120 150 230]/255;c2 = ([120 150 230]+0)/383;c3 = ([120 150 230]+128)/383;patch([0 1 1 0],[0 0 1 1],c1);patch([0 1 1 1-e 1-e 0+e],[0 0 1 1-e 0+e 0+e],c2);patch([0 0 1 1-e 0+e 0+e],[0 1 1 1-e 1-e 0+e],c3);plot([0 1 1 0 0],[0 0 1 1 0]);disp('Weights');
  "IW{1,1}(153,:)'" : Constant  Value=[0.49208453507465821363808800015249289572238922119140625;-0.12775002808200197623733629370690323412418365478515625;-3.21189853551724890934337963699363172054290771484375;-1.189710205898109052213840186595916748046875;-0.38848386976514703849971965610166080296039581298828125;-0.04460953449357467348601602452617953531444072723388671875]
      mask Display: e = 0.06;c1 = [120 150 230]/255;c2 = ([120 150 230]+0)/383;c3 = ([120 150 230]+128)/383;patch([0 1 1 0],[0 0 1 1],c1);patch([0 1 1 1-e 1-e 0+e],[0 0 1 1-e 0+e 0+e],c2);patch([0 0 1 1-e 0+e 0+e],[0 1 1 1-e 1-e 0+e],c3);plot([0 1 1 0 0],[0 0 1 1 0]);disp('Weights');
  "IW{1,1}(154,:)'" : Constant  Value=[-0.4215071133682701809419768324005417525768280029296875;0.31629540536159395092141721761436201632022857666015625;-1.489287162254327778754259270499460399150848388671875;2.27872065300168014090331780607812106609344482421875;-1.6435104536116380558041782933287322521209716796875;1.385346402915233365860103731392882764339447021484375]
      mask Display: e = 0.06;c1 = [120 150 230]/255;c2 = ([120 150 230]+0)/383;c3 = ([120 150 230]+128)/383;patch([0 1 1 0],[0 0 1 1],c1);patch([0 1 1 1-e 1-e 0+e],[0 0 1 1-e 0+e 0+e],c2);patch([0 0 1 1-e 0+e 0+e],[0 1 1 1-e 1-e 0+e],c3);plot([0 1 1 0 0],[0 0 1 1 0]);disp('Weights');
  "IW{1,1}(155,:)'" : Constant  Value=[0.1948496512176222938972358633691328577697277069091796875;1.5320932379684604196512509588501416146755218505859375;-1.0683340270808472372010555773158557713031768798828125;1.91720486504949594319668904063291847705841064453125;-1.1137693580619634214912139213993214070796966552734375;1.6013657296772201288348469461197964847087860107421875]
      mask Display: e = 0.06;c1 = [120 150 230]/255;c2 = ([120 150 230]+0)/383;c3 = ([120 150 230]+128)/383;patch([0 1 1 0],[0 0 1 1],c1);patch([0 1 1 1-e 1-e 0+e],[0 0 1 1-e 0+e 0+e],c2);patch([0 0 1 1-e 0+e 0+e],[0 1 1 1-e 1-e 0+e],c3);plot([0 1 1 0 0],[0 0 1 1 0]);disp('Weights');
  "IW{1,1}(156,:)'" : Constant  Value=[1.5429052657362223310855142699438147246837615966796875;-1.8906066740935667525036478764377534389495849609375;-0.63527596346648695924130834100651554763317108154296875;-1.212205615390997248681514975032769143581390380859375;0.54708394724894848781815426264074631035327911376953125;1.7961358810148742026768786672619171440601348876953125]
      mask Display: e = 0.06;c1 = [120 150 230]/255;c2 = ([120 150 230]+0)/383;c3 = ([120 150 230]+128)/383;patch([0 1 1 0],[0 0 1 1],c1);patch([0 1 1 1-e 1-e 0+e],[0 0 1 1-e 0+e 0+e],c2);patch([0 0 1 1-e 0+e 0+e],[0 1 1 1-e 1-e 0+e],c3);plot([0 1 1 0 0],[0 0 1 1 0]);disp('Weights');
  "IW{1,1}(157,:)'" : Constant  Value=[-0.426877381018563706316371053617331199347972869873046875;-1.8567215485866714885787587263621389865875244140625;2.775714710908702809177839299081824719905853271484375;-0.66694235293821690913063093830714933574199676513671875;0.44411441828389541797150741331279277801513671875;0.3786291035681175198845949125825427472591400146484375]
      mask Display: e = 0.06;c1 = [120 150 230]/255;c2 = ([120 150 230]+0)/383;c3 = ([120 150 230]+128)/383;patch([0 1 1 0],[0 0 1 1],c1);patch([0 1 1 1-e 1-e 0+e],[0 0 1 1-e 0+e 0+e],c2);patch([0 0 1 1-e 0+e 0+e],[0 1 1 1-e 1-e 0+e],c3);plot([0 1 1 0 0],[0 0 1 1 0]);disp('Weights');
  "IW{1,1}(158,:)'" : Constant  Value=[-2.109630905938601141969002128462307155132293701171875;1.7856885489417890777730235640774480998516082763671875;0.00924157087740738215908553598865182721056044101715087890625;-0.75331719239897998452448746320442296564579010009765625;1.327790561208163300221940517076291143894195556640625;1.490575225247259272265409890678711235523223876953125]
      mask Display: e = 0.06;c1 = [120 150 230]/255;c2 = ([120 150 230]+0)/383;c3 = ([120 150 230]+128)/383;patch([0 1 1 0],[0 0 1 1],c1);patch([0 1 1 1-e 1-e 0+e],[0 0 1 1-e 0+e 0+e],c2);patch([0 0 1 1-e 0+e 0+e],[0 1 1 1-e 1-e 0+e],c3);plot([0 1 1 0 0],[0 0 1 1 0]);disp('Weights');
  "IW{1,1}(159,:)'" : Constant  Value=[1.902254363037244377920842453022487461566925048828125;1.4924269184048528646968634348013438284397125244140625;0.5642564259056801478919851433602161705493927001953125;1.373479105486155038562401387025602161884307861328125;0.72904794935601191507856810858356766402721405029296875;1.940380359296527412737987106083892285823822021484375]
      mask Display: e = 0.06;c1 = [120 150 230]/255;c2 = ([120 150 230]+0)/383;c3 = ([120 150 230]+128)/383;patch([0 1 1 0],[0 0 1 1],c1);patch([0 1 1 1-e 1-e 0+e],[0 0 1 1-e 0+e 0+e],c2);patch([0 0 1 1-e 0+e 0+e],[0 1 1 1-e 1-e 0+e],c3);plot([0 1 1 0 0],[0 0 1 1 0]);disp('Weights');
  "IW{1,1}(16,:)'" : Constant  Value=[1.7302896154391493865887241554446518421173095703125;-1.7293881933102357439935303773381747305393218994140625;-1.3631776825220727200616011032252572476863861083984375;-1.4163986498659115742526637404807843267917633056640625;-1.505605761474674952893337831483222544193267822265625;0.06820537133815178509887999780403333716094493865966796875]
      mask Display: e = 0.06;c1 = [120 150 230]/255;c2 = ([120 150 230]+0)/383;c3 = ([120 150 230]+128)/383;patch([0 1 1 0],[0 0 1 1],c1);patch([0 1 1 1-e 1-e 0+e],[0 0 1 1-e 0+e 0+e],c2);patch([0 0 1 1-e 0+e 0+e],[0 1 1 1-e 1-e 0+e],c3);plot([0 1 1 0 0],[0 0 1 1 0]);disp('Weights');
  "IW{1,1}(160,:)'" : Constant  Value=[-1.76634000337539109892759370268322527408599853515625;1.768143094826510886008463785401545464992523193359375;-1.6489907116253068597444553233799524605274200439453125;-1.3522725207735610819526073100860230624675750732421875;0.6538620387597406935498156599351204931735992431640625;0.63302947634451200986660523994942195713520050048828125]
      mask Display: e = 0.06;c1 = [120 150 230]/255;c2 = ([120 150 230]+0)/383;c3 = ([120 150 230]+128)/383;patch([0 1 1 0],[0 0 1 1],c1);patch([0 1 1 1-e 1-e 0+e],[0 0 1 1-e 0+e 0+e],c2);patch([0 0 1 1-e 0+e 0+e],[0 1 1 1-e 1-e 0+e],c3);plot([0 1 1 0 0],[0 0 1 1 0]);disp('Weights');
  "IW{1,1}(161,:)'" : Constant  Value=[0.6726788325524497569318782552727498114109039306640625;-1.00570423801408281860858551226556301116943359375;-1.2068824423437922721547010951326228678226470947265625;1.9852444198073337933152515688561834394931793212890625;0.64769935122349331368951652621035464107990264892578125;-2.241804154588701525341321030282415449619293212890625]
      mask Display: e = 0.06;c1 = [120 150 230]/255;c2 = ([120 150 230]+0)/383;c3 = ([120 150 230]+128)/383;patch([0 1 1 0],[0 0 1 1],c1);patch([0 1 1 1-e 1-e 0+e],[0 0 1 1-e 0+e 0+e],c2);patch([0 0 1 1-e 0+e 0+e],[0 1 1 1-e 1-e 0+e],c3);plot([0 1 1 0 0],[0 0 1 1 0]);disp('Weights');
  "IW{1,1}(162,:)'" : Constant  Value=[1.1042900104737476407734675376559607684612274169921875;1.6514665165600355134500887288595549762248992919921875;1.3460950599548624495582771487534046173095703125;-1.928262261457975856870916686602868139743804931640625;-0.938655153324944979686961232800967991352081298828125;-1.4046473358133597653107926817028783261775970458984375]
      mask Display: e = 0.06;c1 = [120 150 230]/255;c2 = ([120 150 230]+0)/383;c3 = ([120 150 230]+128)/383;patch([0 1 1 0],[0 0 1 1],c1);patch([0 1 1 1-e 1-e 0+e],[0 0 1 1-e 0+e 0+e],c2);patch([0 0 1 1-e 0+e 0+e],[0 1 1 1-e 1-e 0+e],c3);plot([0 1 1 0 0],[0 0 1 1 0]);disp('Weights');
  "IW{1,1}(163,:)'" : Constant  Value=[-1.5218787478527795453686621840461157262325286865234375;1.2760973475511547814420509894262067973613739013671875;-0.0608945458033867403901950865474645979702472686767578125;-2.00227609312392562657123562530614435672760009765625;1.0282963317604594255527672430616803467273712158203125;0.93086102404587556247150814670021645724773406982421875]
      mask Display: e = 0.06;c1 = [120 150 230]/255;c2 = ([120 150 230]+0)/383;c3 = ([120 150 230]+128)/383;patch([0 1 1 0],[0 0 1 1],c1);patch([0 1 1 1-e 1-e 0+e],[0 0 1 1-e 0+e 0+e],c2);patch([0 0 1 1-e 0+e 0+e],[0 1 1 1-e 1-e 0+e],c3);plot([0 1 1 0 0],[0 0 1 1 0]);disp('Weights');
  "IW{1,1}(164,:)'" : Constant  Value=[1.382431321614566943623003680841065943241119384765625;1.605528378530816979719020309858024120330810546875;2.067950569533305582581306225620210170745849609375;-0.293192814598550122173747922715847380459308624267578125;0.07319636710883505037461560505107627250254154205322265625;-1.8279197010062784300998828257434070110321044921875]
      mask Display: e = 0.06;c1 = [120 150 230]/255;c2 = ([120 150 230]+0)/383;c3 = ([120 150 230]+128)/383;patch([0 1 1 0],[0 0 1 1],c1);patch([0 1 1 1-e 1-e 0+e],[0 0 1 1-e 0+e 0+e],c2);patch([0 0 1 1-e 0+e 0+e],[0 1 1 1-e 1-e 0+e],c3);plot([0 1 1 0 0],[0 0 1 1 0]);disp('Weights');
  "IW{1,1}(165,:)'" : Constant  Value=[1.8234402485262466431237271535792388021945953369140625;-0.61788023321938723153579076097230426967144012451171875;0.348040700164764349455737146854517050087451934814453125;1.634795650696454050176953387563116848468780517578125;0.09287382887604840597806088453580741770565509796142578125;2.361192568695267279821337069733999669551849365234375]
      mask Display: e = 0.06;c1 = [120 150 230]/255;c2 = ([120 150 230]+0)/383;c3 = ([120 150 230]+128)/383;patch([0 1 1 0],[0 0 1 1],c1);patch([0 1 1 1-e 1-e 0+e],[0 0 1 1-e 0+e 0+e],c2);patch([0 0 1 1-e 0+e 0+e],[0 1 1 1-e 1-e 0+e],c3);plot([0 1 1 0 0],[0 0 1 1 0]);disp('Weights');
  "IW{1,1}(166,:)'" : Constant  Value=[0.28003800577648407799102869830676354467868804931640625;0.01252437196762586600617961352099882788024842739105224609375;-0.374673715885017966087389140739105641841888427734375;1.59116499382011955532334468443877995014190673828125;-2.6230161960881002158885166863910853862762451171875;1.6288783356417118053371950736618600785732269287109375]
      mask Display: e = 0.06;c1 = [120 150 230]/255;c2 = ([120 150 230]+0)/383;c3 = ([120 150 230]+128)/383;patch([0 1 1 0],[0 0 1 1],c1);patch([0 1 1 1-e 1-e 0+e],[0 0 1 1-e 0+e 0+e],c2);patch([0 0 1 1-e 0+e 0+e],[0 1 1 1-e 1-e 0+e],c3);plot([0 1 1 0 0],[0 0 1 1 0]);disp('Weights');
  "IW{1,1}(167,:)'" : Constant  Value=[0.0938355294422278662924696845948346890509128570556640625;1.3741421497996249012629732533241622149944305419921875;1.7626090790482920045434411804308183491230010986328125;1.5159514580504425129703349739429540932178497314453125;0.88732188566418290776027788524515926837921142578125;1.6594958571336830832620989895076490938663482666015625]
      mask Display: e = 0.06;c1 = [120 150 230]/255;c2 = ([120 150 230]+0)/383;c3 = ([120 150 230]+128)/383;patch([0 1 1 0],[0 0 1 1],c1);patch([0 1 1 1-e 1-e 0+e],[0 0 1 1-e 0+e 0+e],c2);patch([0 0 1 1-e 0+e 0+e],[0 1 1 1-e 1-e 0+e],c3);plot([0 1 1 0 0],[0 0 1 1 0]);disp('Weights');
  "IW{1,1}(168,:)'" : Constant  Value=[1.5339048134539188250613506170338951051235198974609375;0.34420234048195685883086980538791976869106292724609375;0.5255523291097023985685154912061989307403564453125;-1.6911687765016301110421181874698959290981292724609375;-2.1620198307003359872169312438927590847015380859375;-1.0265539236789520405324083185405470430850982666015625]
      mask Display: e = 0.06;c1 = [120 150 230]/255;c2 = ([120 150 230]+0)/383;c3 = ([120 150 230]+128)/383;patch([0 1 1 0],[0 0 1 1],c1);patch([0 1 1 1-e 1-e 0+e],[0 0 1 1-e 0+e 0+e],c2);patch([0 0 1 1-e 0+e 0+e],[0 1 1 1-e 1-e 0+e],c3);plot([0 1 1 0 0],[0 0 1 1 0]);disp('Weights');
  "IW{1,1}(169,:)'" : Constant  Value=[-0.8086427382471950142672767469775862991809844970703125;-1.813343117505640922360043987282551825046539306640625;1.9796410726159658910461303094052709639072418212890625;1.32534047594627057975458228611387312412261962890625;1.223153519097488040046073365374468266963958740234375;0.897187060327319318986383223091252148151397705078125]
      mask Display: e = 0.06;c1 = [120 150 230]/255;c2 = ([120 150 230]+0)/383;c3 = ([120 150 230]+128)/383;patch([0 1 1 0],[0 0 1 1],c1);patch([0 1 1 1-e 1-e 0+e],[0 0 1 1-e 0+e 0+e],c2);patch([0 0 1 1-e 0+e 0+e],[0 1 1 1-e 1-e 0+e],c3);plot([0 1 1 0 0],[0 0 1 1 0]);disp('Weights');
  "IW{1,1}(17,:)'" : Constant  Value=[-0.005489355742431527296343318766957963816821575164794921875;-1.491918369829289492400903327506966888904571533203125;2.4479171315019723209616131498478353023529052734375;-1.057178663097393833680825991905294358730316162109375;0.6169109384288378183924805853166617453098297119140625;-1.167071889030131703890447170124389231204986572265625]
      mask Display: e = 0.06;c1 = [120 150 230]/255;c2 = ([120 150 230]+0)/383;c3 = ([120 150 230]+128)/383;patch([0 1 1 0],[0 0 1 1],c1);patch([0 1 1 1-e 1-e 0+e],[0 0 1 1-e 0+e 0+e],c2);patch([0 0 1 1-e 0+e 0+e],[0 1 1 1-e 1-e 0+e],c3);plot([0 1 1 0 0],[0 0 1 1 0]);disp('Weights');
  "IW{1,1}(170,:)'" : Constant  Value=[2.00044700295793642652597554842941462993621826171875;-0.846731602331223687230021823779679834842681884765625;1.0297335529516453700438205487444065511226654052734375;-0.592145870626422432536628548405133187770843505859375;-1.93919474140215175594903485034592449665069580078125;1.167897774606505123529132106341421604156494140625]
      mask Display: e = 0.06;c1 = [120 150 230]/255;c2 = ([120 150 230]+0)/383;c3 = ([120 150 230]+128)/383;patch([0 1 1 0],[0 0 1 1],c1);patch([0 1 1 1-e 1-e 0+e],[0 0 1 1-e 0+e 0+e],c2);patch([0 0 1 1-e 0+e 0+e],[0 1 1 1-e 1-e 0+e],c3);plot([0 1 1 0 0],[0 0 1 1 0]);disp('Weights');
  "IW{1,1}(171,:)'" : Constant  Value=[2.037520056252544176089713801047764718532562255859375;-1.3789943472650503242249442337197251617908477783203125;-1.4895491193725518552781750258873216807842254638671875;-1.7080966167019340229416002330253832042217254638671875;1.14198788414771623678234391263686120510101318359375;-0.27993560607544887286479706745012663304805755615234375]
      mask Display: e = 0.06;c1 = [120 150 230]/255;c2 = ([120 150 230]+0)/383;c3 = ([120 150 230]+128)/383;patch([0 1 1 0],[0 0 1 1],c1);patch([0 1 1 1-e 1-e 0+e],[0 0 1 1-e 0+e 0+e],c2);patch([0 0 1 1-e 0+e 0+e],[0 1 1 1-e 1-e 0+e],c3);plot([0 1 1 0 0],[0 0 1 1 0]);disp('Weights');
  "IW{1,1}(172,:)'" : Constant  Value=[0.260632504702728196033234553397051058709621429443359375;1.1960225442451328792259346300852485001087188720703125;-1.2795950889846372522384854164556600153446197509765625;2.86566907454303265723183358204551041126251220703125;-0.92119758853303290724312546444707550108432769775390625;-0.427950128734994328372209793087677098810672760009765625]
      mask Display: e = 0.06;c1 = [120 150 230]/255;c2 = ([120 150 230]+0)/383;c3 = ([120 150 230]+128)/383;patch([0 1 1 0],[0 0 1 1],c1);patch([0 1 1 1-e 1-e 0+e],[0 0 1 1-e 0+e 0+e],c2);patch([0 0 1 1-e 0+e 0+e],[0 1 1 1-e 1-e 0+e],c3);plot([0 1 1 0 0],[0 0 1 1 0]);disp('Weights');
  "IW{1,1}(173,:)'" : Constant  Value=[1.5527002599338002308826389707974158227443695068359375;-2.134733347336844833108671082300134003162384033203125;-1.3865265836675815247502896454534493386745452880859375;-1.73186968490525838859639407019130885601043701171875;-0.40353673378598153842489182352437637746334075927734375;0.345282000772171471236759998646448366343975067138671875]
      mask Display: e = 0.06;c1 = [120 150 230]/255;c2 = ([120 150 230]+0)/383;c3 = ([120 150 230]+128)/383;patch([0 1 1 0],[0 0 1 1],c1);patch([0 1 1 1-e 1-e 0+e],[0 0 1 1-e 0+e 0+e],c2);patch([0 0 1 1-e 0+e 0+e],[0 1 1 1-e 1-e 0+e],c3);plot([0 1 1 0 0],[0 0 1 1 0]);disp('Weights');
  "IW{1,1}(174,:)'" : Constant  Value=[-1.2942640367759399300240374941495247185230255126953125;-0.310990719015765859634115031440160237252712249755859375;-0.45102006004629358049129450591863133013248443603515625;-1.4772838127198808511053584879846312105655670166015625;-2.434081082818533303679942036978900432586669921875;1.5010985695779870408017586669302545487880706787109375]
      mask Display: e = 0.06;c1 = [120 150 230]/255;c2 = ([120 150 230]+0)/383;c3 = ([120 150 230]+128)/383;patch([0 1 1 0],[0 0 1 1],c1);patch([0 1 1 1-e 1-e 0+e],[0 0 1 1-e 0+e 0+e],c2);patch([0 0 1 1-e 0+e 0+e],[0 1 1 1-e 1-e 0+e],c3);plot([0 1 1 0 0],[0 0 1 1 0]);disp('Weights');
  "IW{1,1}(175,:)'" : Constant  Value=[-0.2190009349543115824143768577414448373019695281982421875;1.16640768208939871186657910584472119808197021484375;0.1550503084040439072399664155454956926405429840087890625;-2.89364047167004212468555124360136687755584716796875;-1.403176072073021085628852233639918267726898193359375;0.225102626305496322789423402355168946087360382080078125]
      mask Display: e = 0.06;c1 = [120 150 230]/255;c2 = ([120 150 230]+0)/383;c3 = ([120 150 230]+128)/383;patch([0 1 1 0],[0 0 1 1],c1);patch([0 1 1 1-e 1-e 0+e],[0 0 1 1-e 0+e 0+e],c2);patch([0 0 1 1-e 0+e 0+e],[0 1 1 1-e 1-e 0+e],c3);plot([0 1 1 0 0],[0 0 1 1 0]);disp('Weights');
  "IW{1,1}(176,:)'" : Constant  Value=[1.7759419840263948042746733335661701858043670654296875;0.294269388804225207056930457838461734354496002197265625;1.7366636828752783916485213921987451612949371337890625;-1.93777160329804321037272529792971909046173095703125;1.268039631554176427385982606210745871067047119140625;-0.828558742924481617109222497674636542797088623046875]
      mask Display: e = 0.06;c1 = [120 150 230]/255;c2 = ([120 150 230]+0)/383;c3 = ([120 150 230]+128)/383;patch([0 1 1 0],[0 0 1 1],c1);patch([0 1 1 1-e 1-e 0+e],[0 0 1 1-e 0+e 0+e],c2);patch([0 0 1 1-e 0+e 0+e],[0 1 1 1-e 1-e 0+e],c3);plot([0 1 1 0 0],[0 0 1 1 0]);disp('Weights');
  "IW{1,1}(177,:)'" : Constant  Value=[0.81115362499874710255909349143621511757373809814453125;-1.5298562278057590280155864093103446066379547119140625;1.4824850193340359805205252996529452502727508544921875;0.8474182229239153318900434896931983530521392822265625;2.024154516218465982291263571823947131633758544921875;1.4225710321631499510885987547226250171661376953125]
      mask Display: e = 0.06;c1 = [120 150 230]/255;c2 = ([120 150 230]+0)/383;c3 = ([120 150 230]+128)/383;patch([0 1 1 0],[0 0 1 1],c1);patch([0 1 1 1-e 1-e 0+e],[0 0 1 1-e 0+e 0+e],c2);patch([0 0 1 1-e 0+e 0+e],[0 1 1 1-e 1-e 0+e],c3);plot([0 1 1 0 0],[0 0 1 1 0]);disp('Weights');
  "IW{1,1}(178,:)'" : Constant  Value=[-0.262949525124423211241975195662234909832477569580078125;-2.03173711291864567130005525541491806507110595703125;0.418015282047173919455218538132612593472003936767578125;-2.299290683745276897553821982000954449176788330078125;1.1593359488634451537336644832976162433624267578125;1.181482662886802703638977618538774549961090087890625]
      mask Display: e = 0.06;c1 = [120 150 230]/255;c2 = ([120 150 230]+0)/383;c3 = ([120 150 230]+128)/383;patch([0 1 1 0],[0 0 1 1],c1);patch([0 1 1 1-e 1-e 0+e],[0 0 1 1-e 0+e 0+e],c2);patch([0 0 1 1-e 0+e 0+e],[0 1 1 1-e 1-e 0+e],c3);plot([0 1 1 0 0],[0 0 1 1 0]);disp('Weights');
  "IW{1,1}(179,:)'" : Constant  Value=[1.701214470213570084666798720718361437320709228515625;-1.4145118607288462708737597495201043784618377685546875;0.10871696867576093048501917337489430792629718780517578125;2.04054087109495174701123687555082142353057861328125;-1.224352170348764534679730786592699587345123291015625;-1.2029601329569883372272443011752329766750335693359375]
      mask Display: e = 0.06;c1 = [120 150 230]/255;c2 = ([120 150 230]+0)/383;c3 = ([120 150 230]+128)/383;patch([0 1 1 0],[0 0 1 1],c1);patch([0 1 1 1-e 1-e 0+e],[0 0 1 1-e 0+e 0+e],c2);patch([0 0 1 1-e 0+e 0+e],[0 1 1 1-e 1-e 0+e],c3);plot([0 1 1 0 0],[0 0 1 1 0]);disp('Weights');
  "IW{1,1}(18,:)'" : Constant  Value=[1.5632065291107419824356838944368064403533935546875;-1.3400978574545072685708646531566046178340911865234375;-1.192490068267149982972341604181565344333648681640625;-1.095598514476053164656832450418733060359954833984375;1.96879385059787903600181380170397460460662841796875;-0.87499759647899832959438981561106629669666290283203125]
      mask Display: e = 0.06;c1 = [120 150 230]/255;c2 = ([120 150 230]+0)/383;c3 = ([120 150 230]+128)/383;patch([0 1 1 0],[0 0 1 1],c1);patch([0 1 1 1-e 1-e 0+e],[0 0 1 1-e 0+e 0+e],c2);patch([0 0 1 1-e 0+e 0+e],[0 1 1 1-e 1-e 0+e],c3);plot([0 1 1 0 0],[0 0 1 1 0]);disp('Weights');
  "IW{1,1}(180,:)'" : Constant  Value=[-1.0357477305260835986899792260373942553997039794921875;-1.246086323834497466833681755815632641315460205078125;-1.845208274693886263406739089987240731716156005859375;-2.09464005456467017296517951763235032558441162109375;-1.3755821208771543684434845999930985271930694580078125;0.1435073858986119776925960422886419110000133514404296875]
      mask Display: e = 0.06;c1 = [120 150 230]/255;c2 = ([120 150 230]+0)/383;c3 = ([120 150 230]+128)/383;patch([0 1 1 0],[0 0 1 1],c1);patch([0 1 1 1-e 1-e 0+e],[0 0 1 1-e 0+e 0+e],c2);patch([0 0 1 1-e 0+e 0+e],[0 1 1 1-e 1-e 0+e],c3);plot([0 1 1 0 0],[0 0 1 1 0]);disp('Weights');
  "IW{1,1}(181,:)'" : Constant  Value=[-0.11717595813460779385906107563641853630542755126953125;2.19093150947058834532299442798830568790435791015625;0.956581138628817218005906397593207657337188720703125;-0.24877304659055343716289598887669853866100311279296875;1.8093074370765507286051843038876540958881378173828125;-1.7410903739841874227067819447256624698638916015625]
      mask Display: e = 0.06;c1 = [120 150 230]/255;c2 = ([120 150 230]+0)/383;c3 = ([120 150 230]+128)/383;patch([0 1 1 0],[0 0 1 1],c1);patch([0 1 1 1-e 1-e 0+e],[0 0 1 1-e 0+e 0+e],c2);patch([0 0 1 1-e 0+e 0+e],[0 1 1 1-e 1-e 0+e],c3);plot([0 1 1 0 0],[0 0 1 1 0]);disp('Weights');
  "IW{1,1}(182,:)'" : Constant  Value=[-0.221358752660881619167554390514851547777652740478515625;1.2600457289998174825740306914667598903179168701171875;0.5167508108274143641125419890158809721469879150390625;1.1627938490982441255283674763632006943225860595703125;-1.761231546590322327716648942441679537296295166015625;-1.8787090241064852147445662922109477221965789794921875]
      mask Display: e = 0.06;c1 = [120 150 230]/255;c2 = ([120 150 230]+0)/383;c3 = ([120 150 230]+128)/383;patch([0 1 1 0],[0 0 1 1],c1);patch([0 1 1 1-e 1-e 0+e],[0 0 1 1-e 0+e 0+e],c2);patch([0 0 1 1-e 0+e 0+e],[0 1 1 1-e 1-e 0+e],c3);plot([0 1 1 0 0],[0 0 1 1 0]);disp('Weights');
  "IW{1,1}(183,:)'" : Constant  Value=[-0.84572790225453076118355966173112392425537109375;-1.4656676812313509383756127135711722075939178466796875;1.2630383160251088536796260086703114211559295654296875;1.9963474793361968284699514697422273457050323486328125;1.6367752905749328729001490501104854047298431396484375;0.838618406960719209308763311128132045269012451171875]
      mask Display: e = 0.06;c1 = [120 150 230]/255;c2 = ([120 150 230]+0)/383;c3 = ([120 150 230]+128)/383;patch([0 1 1 0],[0 0 1 1],c1);patch([0 1 1 1-e 1-e 0+e],[0 0 1 1-e 0+e 0+e],c2);patch([0 0 1 1-e 0+e 0+e],[0 1 1 1-e 1-e 0+e],c3);plot([0 1 1 0 0],[0 0 1 1 0]);disp('Weights');
  "IW{1,1}(184,:)'" : Constant  Value=[1.4970991905002148936176809002063237130641937255859375;1.5157752848167878045870793357607908546924591064453125;1.6395857423213027193042989893001504242420196533203125;-1.00928136002138302274033776484429836273193359375;0.129351091816574725879007701223599724471569061279296875;-1.9330447107558790253989400298451073467731475830078125]
      mask Display: e = 0.06;c1 = [120 150 230]/255;c2 = ([120 150 230]+0)/383;c3 = ([120 150 230]+128)/383;patch([0 1 1 0],[0 0 1 1],c1);patch([0 1 1 1-e 1-e 0+e],[0 0 1 1-e 0+e 0+e],c2);patch([0 0 1 1-e 0+e 0+e],[0 1 1 1-e 1-e 0+e],c3);plot([0 1 1 0 0],[0 0 1 1 0]);disp('Weights');
  "IW{1,1}(185,:)'" : Constant  Value=[1.472866437664254846140465815551578998565673828125;-0.3270490038565785351210024600732140243053436279296875;-1.5482260708738893040248285615234635770320892333984375;1.802755297827359104445577031583525240421295166015625;1.423438405781123794469067433965392410755157470703125;-1.297548315459566392604529028176330029964447021484375]
      mask Display: e = 0.06;c1 = [120 150 230]/255;c2 = ([120 150 230]+0)/383;c3 = ([120 150 230]+128)/383;patch([0 1 1 0],[0 0 1 1],c1);patch([0 1 1 1-e 1-e 0+e],[0 0 1 1-e 0+e 0+e],c2);patch([0 0 1 1-e 0+e 0+e],[0 1 1 1-e 1-e 0+e],c3);plot([0 1 1 0 0],[0 0 1 1 0]);disp('Weights');
  "IW{1,1}(186,:)'" : Constant  Value=[-0.79883212760156829812530077106202952563762664794921875;1.4051265239059602674132065658341161906719207763671875;1.0233384446733364558923540243995375931262969970703125;1.718116298209971137822549280826933681964874267578125;0.320589804476596851312564240288338623940944671630859375;2.3135486975211190241452641203068196773529052734375]
      mask Display: e = 0.06;c1 = [120 150 230]/255;c2 = ([120 150 230]+0)/383;c3 = ([120 150 230]+128)/383;patch([0 1 1 0],[0 0 1 1],c1);patch([0 1 1 1-e 1-e 0+e],[0 0 1 1-e 0+e 0+e],c2);patch([0 0 1 1-e 0+e 0+e],[0 1 1 1-e 1-e 0+e],c3);plot([0 1 1 0 0],[0 0 1 1 0]);disp('Weights');
  "IW{1,1}(187,:)'" : Constant  Value=[2.22762045061896873932028029230423271656036376953125;-0.971398115098014880430810080724768340587615966796875;-1.500248322152097468773490618332289159297943115234375;-1.9729353879384066150493026725598610937595367431640625;0.09297738254103556088114856947868247516453266143798828125;0.42215696060550145229939289492904208600521087646484375]
      mask Display: e = 0.06;c1 = [120 150 230]/255;c2 = ([120 150 230]+0)/383;c3 = ([120 150 230]+128)/383;patch([0 1 1 0],[0 0 1 1],c1);patch([0 1 1 1-e 1-e 0+e],[0 0 1 1-e 0+e 0+e],c2);patch([0 0 1 1-e 0+e 0+e],[0 1 1 1-e 1-e 0+e],c3);plot([0 1 1 0 0],[0 0 1 1 0]);disp('Weights');
  "IW{1,1}(188,:)'" : Constant  Value=[-0.88561637243580981770918469919706694781780242919921875;0.308803588403619266866684256456210277974605560302734375;2.00670720624670639864461918477900326251983642578125;-1.859689052599113434638411490595899522304534912109375;1.7808393685753574064989379621692933142185211181640625;0.90088608279449056137622164897038601338863372802734375]
      mask Display: e = 0.06;c1 = [120 150 230]/255;c2 = ([120 150 230]+0)/383;c3 = ([120 150 230]+128)/383;patch([0 1 1 0],[0 0 1 1],c1);patch([0 1 1 1-e 1-e 0+e],[0 0 1 1-e 0+e 0+e],c2);patch([0 0 1 1-e 0+e 0+e],[0 1 1 1-e 1-e 0+e],c3);plot([0 1 1 0 0],[0 0 1 1 0]);disp('Weights');
  "IW{1,1}(189,:)'" : Constant  Value=[1.310898061619692356316591030918061733245849609375;1.6388916594826794526085222969413734972476959228515625;1.49536261134549075535460360697470605373382568359375;-0.85979895594227062627368241010117344558238983154296875;-1.1763535100704842761842883192002773284912109375;1.6741611440444330582977272570133209228515625]
      mask Display: e = 0.06;c1 = [120 150 230]/255;c2 = ([120 150 230]+0)/383;c3 = ([120 150 230]+128)/383;patch([0 1 1 0],[0 0 1 1],c1);patch([0 1 1 1-e 1-e 0+e],[0 0 1 1-e 0+e 0+e],c2);patch([0 0 1 1-e 0+e 0+e],[0 1 1 1-e 1-e 0+e],c3);plot([0 1 1 0 0],[0 0 1 1 0]);disp('Weights');
  "IW{1,1}(19,:)'" : Constant  Value=[2.452901756227767737783551638131029903888702392578125;0.96155796162006412775014041471877135336399078369140625;0.41401680988201861044473162110080011188983917236328125;-0.1765013702928645844547617116404580883681774139404296875;1.24723096617993345347485956153832376003265380859375;-2.0721887322793062224945970228873193264007568359375]
      mask Display: e = 0.06;c1 = [120 150 230]/255;c2 = ([120 150 230]+0)/383;c3 = ([120 150 230]+128)/383;patch([0 1 1 0],[0 0 1 1],c1);patch([0 1 1 1-e 1-e 0+e],[0 0 1 1-e 0+e 0+e],c2);patch([0 0 1 1-e 0+e 0+e],[0 1 1 1-e 1-e 0+e],c3);plot([0 1 1 0 0],[0 0 1 1 0]);disp('Weights');
  "IW{1,1}(190,:)'" : Constant  Value=[-1.801363776334323318906172062270343303680419921875;0.53616928518241524503906703102984465658664703369140625;1.735480107761147916534127944032661616802215576171875;-1.7614133672332961122464212166960351169109344482421875;-1.1979756087006772080627570176147855818271636962890625;1.44288015296377647445069669629447162151336669921875]
      mask Display: e = 0.06;c1 = [120 150 230]/255;c2 = ([120 150 230]+0)/383;c3 = ([120 150 230]+128)/383;patch([0 1 1 0],[0 0 1 1],c1);patch([0 1 1 1-e 1-e 0+e],[0 0 1 1-e 0+e 0+e],c2);patch([0 0 1 1-e 0+e 0+e],[0 1 1 1-e 1-e 0+e],c3);plot([0 1 1 0 0],[0 0 1 1 0]);disp('Weights');
  "IW{1,1}(191,:)'" : Constant  Value=[1.668215398475793254107202301383949816226959228515625;1.496702355588922284113095884094946086406707763671875;-1.805199776186109605902174735092557966709136962890625;1.5177930668726851148875311992014758288860321044921875;-1.0892839586138280960625479565351270139217376708984375;0.9798566255040828121281037965673021972179412841796875]
      mask Display: e = 0.06;c1 = [120 150 230]/255;c2 = ([120 150 230]+0)/383;c3 = ([120 150 230]+128)/383;patch([0 1 1 0],[0 0 1 1],c1);patch([0 1 1 1-e 1-e 0+e],[0 0 1 1-e 0+e 0+e],c2);patch([0 0 1 1-e 0+e 0+e],[0 1 1 1-e 1-e 0+e],c3);plot([0 1 1 0 0],[0 0 1 1 0]);disp('Weights');
  "IW{1,1}(192,:)'" : Constant  Value=[1.8191161698083988529361931796302087604999542236328125;-0.7710748462874621456109025530167855322360992431640625;0.257746071315022307057773787164478562772274017333984375;-2.21663502322562777635539532639086246490478515625;1.32441879378441029757595970295369625091552734375;1.3284356840920954478946214294410310685634613037109375]
      mask Display: e = 0.06;c1 = [120 150 230]/255;c2 = ([120 150 230]+0)/383;c3 = ([120 150 230]+128)/383;patch([0 1 1 0],[0 0 1 1],c1);patch([0 1 1 1-e 1-e 0+e],[0 0 1 1-e 0+e 0+e],c2);patch([0 0 1 1-e 0+e 0+e],[0 1 1 1-e 1-e 0+e],c3);plot([0 1 1 0 0],[0 0 1 1 0]);disp('Weights');
  "IW{1,1}(193,:)'" : Constant  Value=[0.017122463583895110306176690073698409833014011383056640625;-0.604343077217572410830825901939533650875091552734375;-1.256978366977978822660588775761425495147705078125;2.602842102311939687098174545099027454853057861328125;0.5041494234935404161745964302099309861660003662109375;-1.5433986546144395912705249429563991725444793701171875]
      mask Display: e = 0.06;c1 = [120 150 230]/255;c2 = ([120 150 230]+0)/383;c3 = ([120 150 230]+128)/383;patch([0 1 1 0],[0 0 1 1],c1);patch([0 1 1 1-e 1-e 0+e],[0 0 1 1-e 0+e 0+e],c2);patch([0 0 1 1-e 0+e 0+e],[0 1 1 1-e 1-e 0+e],c3);plot([0 1 1 0 0],[0 0 1 1 0]);disp('Weights');
  "IW{1,1}(194,:)'" : Constant  Value=[-2.132927968445128552588130332878790795803070068359375;0.9432896547028588596361942109069786965847015380859375;-1.8875347865294356264342923168442212045192718505859375;-1.778712778548842354808812160626985132694244384765625;0.50384142208576576660306045596371404826641082763671875;-0.2429245054914697388159794400053215213119983673095703125]
      mask Display: e = 0.06;c1 = [120 150 230]/255;c2 = ([120 150 230]+0)/383;c3 = ([120 150 230]+128)/383;patch([0 1 1 0],[0 0 1 1],c1);patch([0 1 1 1-e 1-e 0+e],[0 0 1 1-e 0+e 0+e],c2);patch([0 0 1 1-e 0+e 0+e],[0 1 1 1-e 1-e 0+e],c3);plot([0 1 1 0 0],[0 0 1 1 0]);disp('Weights');
  "IW{1,1}(195,:)'" : Constant  Value=[1.1367232606977413222892892008530907332897186279296875;2.39041820373336211247305982396937906742095947265625;-1.2194483878463968640204484472633339464664459228515625;-0.74012116427745422431172528376919217407703399658203125;1.0370062246316995580031061763293109834194183349609375;-1.445401898705347409901378341601230204105377197265625]
      mask Display: e = 0.06;c1 = [120 150 230]/255;c2 = ([120 150 230]+0)/383;c3 = ([120 150 230]+128)/383;patch([0 1 1 0],[0 0 1 1],c1);patch([0 1 1 1-e 1-e 0+e],[0 0 1 1-e 0+e 0+e],c2);patch([0 0 1 1-e 0+e 0+e],[0 1 1 1-e 1-e 0+e],c3);plot([0 1 1 0 0],[0 0 1 1 0]);disp('Weights');
  "IW{1,1}(196,:)'" : Constant  Value=[-0.6114361608207377063450849163928069174289703369140625;-0.005146594284178323229494989021759465686045587062835693359375;-1.9491460132331288601648111580288968980312347412109375;-1.20187091289669734095468811574392020702362060546875;-2.092649434475525094256909142131917178630828857421875;-1.6256547289481428908430871160817332565784454345703125]
      mask Display: e = 0.06;c1 = [120 150 230]/255;c2 = ([120 150 230]+0)/383;c3 = ([120 150 230]+128)/383;patch([0 1 1 0],[0 0 1 1],c1);patch([0 1 1 1-e 1-e 0+e],[0 0 1 1-e 0+e 0+e],c2);patch([0 0 1 1-e 0+e 0+e],[0 1 1 1-e 1-e 0+e],c3);plot([0 1 1 0 0],[0 0 1 1 0]);disp('Weights');
  "IW{1,1}(197,:)'" : Constant  Value=[1.9140150111094322848970250561251305043697357177734375;-0.7312034358101922038031261763535439968109130859375;-1.3662689054945957867204242575098760426044464111328125;0.58756915765710593380077852998510934412479400634765625;2.333712225160908371179857567767612636089324951171875;-0.99249301179533799821541606434038840234279632568359375]
      mask Display: e = 0.06;c1 = [120 150 230]/255;c2 = ([120 150 230]+0)/383;c3 = ([120 150 230]+128)/383;patch([0 1 1 0],[0 0 1 1],c1);patch([0 1 1 1-e 1-e 0+e],[0 0 1 1-e 0+e 0+e],c2);patch([0 0 1 1-e 0+e 0+e],[0 1 1 1-e 1-e 0+e],c3);plot([0 1 1 0 0],[0 0 1 1 0]);disp('Weights');
  "IW{1,1}(198,:)'" : Constant  Value=[-0.3418453589438008588530237830127589404582977294921875;0.54439434743706105468419309545424766838550567626953125;2.437965064049400165657743855263106524944305419921875;0.40293727429620040947355619209702126681804656982421875;-2.04743841283180660894913671654649078845977783203125;1.08009946016262947665609317482449114322662353515625]
      mask Display: e = 0.06;c1 = [120 150 230]/255;c2 = ([120 150 230]+0)/383;c3 = ([120 150 230]+128)/383;patch([0 1 1 0],[0 0 1 1],c1);patch([0 1 1 1-e 1-e 0+e],[0 0 1 1-e 0+e 0+e],c2);patch([0 0 1 1-e 0+e 0+e],[0 1 1 1-e 1-e 0+e],c3);plot([0 1 1 0 0],[0 0 1 1 0]);disp('Weights');
  "IW{1,1}(199,:)'" : Constant  Value=[0.394245035098662210959474805349600501358509063720703125;1.6373512187027372544179115720908157527446746826171875;1.4797233889563325970328833136591129004955291748046875;-1.03643999422008459276867142762057483196258544921875;2.3515960269574929242253347183577716350555419921875;-0.2421289457005978140724522518212324939668178558349609375]
      mask Display: e = 0.06;c1 = [120 150 230]/255;c2 = ([120 150 230]+0)/383;c3 = ([120 150 230]+128)/383;patch([0 1 1 0],[0 0 1 1],c1);patch([0 1 1 1-e 1-e 0+e],[0 0 1 1-e 0+e 0+e],c2);patch([0 0 1 1-e 0+e 0+e],[0 1 1 1-e 1-e 0+e],c3);plot([0 1 1 0 0],[0 0 1 1 0]);disp('Weights');
  "IW{1,1}(2,:)'" : Constant  Value=[-1.616415708951979279817123824614100158214569091796875;-1.1294443107311342711085444534546695649623870849609375;-1.62225280755765677298541049822233617305755615234375;0.9645188239586985901041771285235881805419921875;1.1773980031868529483318752681952901184558868408203125;1.631703357973727452900902790133841335773468017578125]
      mask Display: e = 0.06;c1 = [120 150 230]/255;c2 = ([120 150 230]+0)/383;c3 = ([120 150 230]+128)/383;patch([0 1 1 0],[0 0 1 1],c1);patch([0 1 1 1-e 1-e 0+e],[0 0 1 1-e 0+e 0+e],c2);patch([0 0 1 1-e 0+e 0+e],[0 1 1 1-e 1-e 0+e],c3);plot([0 1 1 0 0],[0 0 1 1 0]);disp('Weights');
  "IW{1,1}(20,:)'" : Constant  Value=[1.462969981172923095158466821885667741298675537109375;0.58876049773030658673889092824538238346576690673828125;0.7675291281729095249630745456670410931110382080078125;0.74307234972066160683112912010983563959598541259765625;-2.141153864056182243302828283049166202545166015625;1.82876593089481698228837558417581021785736083984375]
      mask Display: e = 0.06;c1 = [120 150 230]/255;c2 = ([120 150 230]+0)/383;c3 = ([120 150 230]+128)/383;patch([0 1 1 0],[0 0 1 1],c1);patch([0 1 1 1-e 1-e 0+e],[0 0 1 1-e 0+e 0+e],c2);patch([0 0 1 1-e 0+e 0+e],[0 1 1 1-e 1-e 0+e],c3);plot([0 1 1 0 0],[0 0 1 1 0]);disp('Weights');
  "IW{1,1}(200,:)'" : Constant  Value=[-0.63705177644893085098232177188037894666194915771484375;-0.351064253679278459596702077760710380971431732177734375;-2.34131667072303972787494785734452307224273681640625;1.28233272873880377318300816114060580730438232421875;-1.9505229211054861959695472251041792333126068115234375;-0.1110745309870048436184930551462457515299320220947265625]
      mask Display: e = 0.06;c1 = [120 150 230]/255;c2 = ([120 150 230]+0)/383;c3 = ([120 150 230]+128)/383;patch([0 1 1 0],[0 0 1 1],c1);patch([0 1 1 1-e 1-e 0+e],[0 0 1 1-e 0+e 0+e],c2);patch([0 0 1 1-e 0+e 0+e],[0 1 1 1-e 1-e 0+e],c3);plot([0 1 1 0 0],[0 0 1 1 0]);disp('Weights');
  "IW{1,1}(201,:)'" : Constant  Value=[0.7566461528970267469418331529595889151096343994140625;-1.0603052120179052852932954920106567442417144775390625;2.1525748388324092985612878692336380481719970703125;-1.88446712622462886344010257744230329990386962890625;1.3990923775924368754886017995886504650115966796875;-1.08778952364815761910676883417181670665740966796875]
      mask Display: e = 0.06;c1 = [120 150 230]/255;c2 = ([120 150 230]+0)/383;c3 = ([120 150 230]+128)/383;patch([0 1 1 0],[0 0 1 1],c1);patch([0 1 1 1-e 1-e 0+e],[0 0 1 1-e 0+e 0+e],c2);patch([0 0 1 1-e 0+e 0+e],[0 1 1 1-e 1-e 0+e],c3);plot([0 1 1 0 0],[0 0 1 1 0]);disp('Weights');
  "IW{1,1}(202,:)'" : Constant  Value=[-0.9090557451564134083810131414793431758880615234375;-0.9038033342030409311718130993540398776531219482421875;2.64230876544299864150389112182892858982086181640625;-1.3447696748422124368715913078631274402141571044921875;1.098185496298234031797846910194493830204010009765625;0.6788670162489947035311388390255160629749298095703125]
      mask Display: e = 0.06;c1 = [120 150 230]/255;c2 = ([120 150 230]+0)/383;c3 = ([120 150 230]+128)/383;patch([0 1 1 0],[0 0 1 1],c1);patch([0 1 1 1-e 1-e 0+e],[0 0 1 1-e 0+e 0+e],c2);patch([0 0 1 1-e 0+e 0+e],[0 1 1 1-e 1-e 0+e],c3);plot([0 1 1 0 0],[0 0 1 1 0]);disp('Weights');
  "IW{1,1}(203,:)'" : Constant  Value=[1.798530616240921364834548512590117752552032470703125;-1.4775343855091052081007774177123792469501495361328125;-1.3810077325781706658602843162952922284603118896484375;1.5925606780397305595187162907677702605724334716796875;1.252456003997191924526077855261974036693572998046875;0.9764534074907944560806072331615723669528961181640625]
      mask Display: e = 0.06;c1 = [120 150 230]/255;c2 = ([120 150 230]+0)/383;c3 = ([120 150 230]+128)/383;patch([0 1 1 0],[0 0 1 1],c1);patch([0 1 1 1-e 1-e 0+e],[0 0 1 1-e 0+e 0+e],c2);patch([0 0 1 1-e 0+e 0+e],[0 1 1 1-e 1-e 0+e],c3);plot([0 1 1 0 0],[0 0 1 1 0]);disp('Weights');
  "IW{1,1}(204,:)'" : Constant  Value=[1.509559470818476523135132083552889525890350341796875;-0.62107152642128216069039581270772032439708709716796875;-0.96599165781246265627402181053184904158115386962890625;1.7954555021314935192577877387520857155323028564453125;1.0468662012440856923234377973130904138088226318359375;-1.90256547656382934974317322485148906707763671875]
      mask Display: e = 0.06;c1 = [120 150 230]/255;c2 = ([120 150 230]+0)/383;c3 = ([120 150 230]+128)/383;patch([0 1 1 0],[0 0 1 1],c1);patch([0 1 1 1-e 1-e 0+e],[0 0 1 1-e 0+e 0+e],c2);patch([0 0 1 1-e 0+e 0+e],[0 1 1 1-e 1-e 0+e],c3);plot([0 1 1 0 0],[0 0 1 1 0]);disp('Weights');
  "IW{1,1}(205,:)'" : Constant  Value=[1.3851262186243145091424366910359822213649749755859375;0.78442139270404409590042860145331360399723052978515625;1.031980173926748012291909617488272488117218017578125;-1.9878238086561192954349053252371959388256072998046875;1.84278029570570112127825268544256687164306640625;1.7024598311534957506552245831699110567569732666015625]
      mask Display: e = 0.06;c1 = [120 150 230]/255;c2 = ([120 150 230]+0)/383;c3 = ([120 150 230]+128)/383;patch([0 1 1 0],[0 0 1 1],c1);patch([0 1 1 1-e 1-e 0+e],[0 0 1 1-e 0+e 0+e],c2);patch([0 0 1 1-e 0+e 0+e],[0 1 1 1-e 1-e 0+e],c3);plot([0 1 1 0 0],[0 0 1 1 0]);disp('Weights');
  "IW{1,1}(206,:)'" : Constant  Value=[-0.94897071308789426868912642021314240992069244384765625;0.0701635155357752948734884057557792402803897857666015625;-2.057675603588080104344726350973360240459442138671875;2.112980923897243901166120849666185677051544189453125;-1.36919867521067661897404832416214048862457275390625;0.5551118807322488191147158431704156100749969482421875]
      mask Display: e = 0.06;c1 = [120 150 230]/255;c2 = ([120 150 230]+0)/383;c3 = ([120 150 230]+128)/383;patch([0 1 1 0],[0 0 1 1],c1);patch([0 1 1 1-e 1-e 0+e],[0 0 1 1-e 0+e 0+e],c2);patch([0 0 1 1-e 0+e 0+e],[0 1 1 1-e 1-e 0+e],c3);plot([0 1 1 0 0],[0 0 1 1 0]);disp('Weights');
  "IW{1,1}(207,:)'" : Constant  Value=[1.1883515911277096055442825672798790037631988525390625;0.78739854444811940847870346260606311261653900146484375;-1.179988137955705784776228028931654989719390869140625;-0.1947715583943859518623042959006852470338344573974609375;-1.650562210892228431902140073361806571483612060546875;2.008228059958179212429740800871513783931732177734375]
      mask Display: e = 0.06;c1 = [120 150 230]/255;c2 = ([120 150 230]+0)/383;c3 = ([120 150 230]+128)/383;patch([0 1 1 0],[0 0 1 1],c1);patch([0 1 1 1-e 1-e 0+e],[0 0 1 1-e 0+e 0+e],c2);patch([0 0 1 1-e 0+e 0+e],[0 1 1 1-e 1-e 0+e],c3);plot([0 1 1 0 0],[0 0 1 1 0]);disp('Weights');
  "IW{1,1}(208,:)'" : Constant  Value=[-0.6026304182828285949113933384069241583347320556640625;-1.0664293683934527035006567530217580497264862060546875;-1.1821256663211456849893465914647094905376434326171875;0.02418091168977769267467436975493910722434520721435546875;-2.22355596025103974255898720002733170986175537109375;1.9762927687746778548927295560133643448352813720703125]
      mask Display: e = 0.06;c1 = [120 150 230]/255;c2 = ([120 150 230]+0)/383;c3 = ([120 150 230]+128)/383;patch([0 1 1 0],[0 0 1 1],c1);patch([0 1 1 1-e 1-e 0+e],[0 0 1 1-e 0+e 0+e],c2);patch([0 0 1 1-e 0+e 0+e],[0 1 1 1-e 1-e 0+e],c3);plot([0 1 1 0 0],[0 0 1 1 0]);disp('Weights');
  "IW{1,1}(209,:)'" : Constant  Value=[1.292326633623141152185098690097220242023468017578125;1.1001781468715499112676070581073872745037078857421875;1.1817024172230616851919648979674093425273895263671875;0.5889386744648259508494447800330817699432373046875;2.03591562646506840650317826657555997371673583984375;-1.7528943503369325274121592883602716028690338134765625]
      mask Display: e = 0.06;c1 = [120 150 230]/255;c2 = ([120 150 230]+0)/383;c3 = ([120 150 230]+128)/383;patch([0 1 1 0],[0 0 1 1],c1);patch([0 1 1 1-e 1-e 0+e],[0 0 1 1-e 0+e 0+e],c2);patch([0 0 1 1-e 0+e 0+e],[0 1 1 1-e 1-e 0+e],c3);plot([0 1 1 0 0],[0 0 1 1 0]);disp('Weights');
  "IW{1,1}(21,:)'" : Constant  Value=[-0.345660969341652968278566504523041658103466033935546875;2.58214158177433805718692383379675447940826416015625;-0.0581906032559310892882109556012437678873538970947265625;-1.284035349835995543088529302622191607952117919921875;-0.207789235728200349928584955705446191132068634033203125;-1.71097044140582266180672377231530845165252685546875]
      mask Display: e = 0.06;c1 = [120 150 230]/255;c2 = ([120 150 230]+0)/383;c3 = ([120 150 230]+128)/383;patch([0 1 1 0],[0 0 1 1],c1);patch([0 1 1 1-e 1-e 0+e],[0 0 1 1-e 0+e 0+e],c2);patch([0 0 1 1-e 0+e 0+e],[0 1 1 1-e 1-e 0+e],c3);plot([0 1 1 0 0],[0 0 1 1 0]);disp('Weights');
  "IW{1,1}(210,:)'" : Constant  Value=[1.2945248413115029162412383811897598206996917724609375;2.007771974900429245991517746006138622760772705078125;0.21169453653223702094265945561346597969532012939453125;0.16185867834566247669414451593183912336826324462890625;1.853119556166209047631809880840592086315155029296875;-0.3519134829402259523334350888035260140895843505859375]
      mask Display: e = 0.06;c1 = [120 150 230]/255;c2 = ([120 150 230]+0)/383;c3 = ([120 150 230]+128)/383;patch([0 1 1 0],[0 0 1 1],c1);patch([0 1 1 1-e 1-e 0+e],[0 0 1 1-e 0+e 0+e],c2);patch([0 0 1 1-e 0+e 0+e],[0 1 1 1-e 1-e 0+e],c3);plot([0 1 1 0 0],[0 0 1 1 0]);disp('Weights');
  "IW{1,1}(211,:)'" : Constant  Value=[1.892058208014297360222144561703316867351531982421875;0.74665150317708761651402937786770053207874298095703125;-1.36443060795185733269363481667824089527130126953125;1.8265978961514266476484635859378613531589508056640625;1.61081027904355789104329232941381633281707763671875;-0.67679279410817583251258611198863945901393890380859375]
      mask Display: e = 0.06;c1 = [120 150 230]/255;c2 = ([120 150 230]+0)/383;c3 = ([120 150 230]+128)/383;patch([0 1 1 0],[0 0 1 1],c1);patch([0 1 1 1-e 1-e 0+e],[0 0 1 1-e 0+e 0+e],c2);patch([0 0 1 1-e 0+e 0+e],[0 1 1 1-e 1-e 0+e],c3);plot([0 1 1 0 0],[0 0 1 1 0]);disp('Weights');
  "IW{1,1}(212,:)'" : Constant  Value=[-1.66546542578679801493990453309379518032073974609375;-1.8141460729657448158747001798474229872226715087890625;-1.6753793331040307545976020264788530766963958740234375;0.400049120890783260762191275716759264469146728515625;0.85879512372468702618988345420802943408489227294921875;-1.6999919009965573923892634411458857357501983642578125]
      mask Display: e = 0.06;c1 = [120 150 230]/255;c2 = ([120 150 230]+0)/383;c3 = ([120 150 230]+128)/383;patch([0 1 1 0],[0 0 1 1],c1);patch([0 1 1 1-e 1-e 0+e],[0 0 1 1-e 0+e 0+e],c2);patch([0 0 1 1-e 0+e 0+e],[0 1 1 1-e 1-e 0+e],c3);plot([0 1 1 0 0],[0 0 1 1 0]);disp('Weights');
  "IW{1,1}(213,:)'" : Constant  Value=[-1.5292019568748174140893070216407068073749542236328125;0.433188369366115655356708202816662378609180450439453125;-0.51286689592992207309407604043371975421905517578125;0.72230185886147590945682850360753946006298065185546875;-1.9679999925094493473665124838589690625667572021484375;2.1897539007929793797302409075200557708740234375]
      mask Display: e = 0.06;c1 = [120 150 230]/255;c2 = ([120 150 230]+0)/383;c3 = ([120 150 230]+128)/383;patch([0 1 1 0],[0 0 1 1],c1);patch([0 1 1 1-e 1-e 0+e],[0 0 1 1-e 0+e 0+e],c2);patch([0 0 1 1-e 0+e 0+e],[0 1 1 1-e 1-e 0+e],c3);plot([0 1 1 0 0],[0 0 1 1 0]);disp('Weights');
  "IW{1,1}(214,:)'" : Constant  Value=[-0.6900010191659420311083295018761418759822845458984375;-0.9976473982769038517659510034718550741672515869140625;-2.533193676260598437011140049435198307037353515625;-1.0729963601083805091462863856577314436435699462890625;1.019636389228790296357374245417304337024688720703125;-1.3011718987962253013535018908441998064517974853515625]
      mask Display: e = 0.06;c1 = [120 150 230]/255;c2 = ([120 150 230]+0)/383;c3 = ([120 150 230]+128)/383;patch([0 1 1 0],[0 0 1 1],c1);patch([0 1 1 1-e 1-e 0+e],[0 0 1 1-e 0+e 0+e],c2);patch([0 0 1 1-e 0+e 0+e],[0 1 1 1-e 1-e 0+e],c3);plot([0 1 1 0 0],[0 0 1 1 0]);disp('Weights');
  "IW{1,1}(215,:)'" : Constant  Value=[1.58138817532090936168742700829170644283294677734375;0.05030994994543731835268118857129593379795551300048828125;2.048240481873010221391950835823081433773040771484375;2.24961971619618328332990131457336246967315673828125;-0.439554703471611685205999719983083195984363555908203125;-0.4602071341014510874600773604470305144786834716796875]
      mask Display: e = 0.06;c1 = [120 150 230]/255;c2 = ([120 150 230]+0)/383;c3 = ([120 150 230]+128)/383;patch([0 1 1 0],[0 0 1 1],c1);patch([0 1 1 1-e 1-e 0+e],[0 0 1 1-e 0+e 0+e],c2);patch([0 0 1 1-e 0+e 0+e],[0 1 1 1-e 1-e 0+e],c3);plot([0 1 1 0 0],[0 0 1 1 0]);disp('Weights');
  "IW{1,1}(216,:)'" : Constant  Value=[-0.34808068168366756989229315877310000360012054443359375;-0.389785789343835842313268358338973484933376312255859375;-1.791712780071231581047186409705318510532379150390625;1.7375283232422427115437812972231768071651458740234375;1.030130714255743651364127799752168357372283935546875;1.79592022464391032343655751901678740978240966796875]
      mask Display: e = 0.06;c1 = [120 150 230]/255;c2 = ([120 150 230]+0)/383;c3 = ([120 150 230]+128)/383;patch([0 1 1 0],[0 0 1 1],c1);patch([0 1 1 1-e 1-e 0+e],[0 0 1 1-e 0+e 0+e],c2);patch([0 0 1 1-e 0+e 0+e],[0 1 1 1-e 1-e 0+e],c3);plot([0 1 1 0 0],[0 0 1 1 0]);disp('Weights');
  "IW{1,1}(217,:)'" : Constant  Value=[-1.67491168186440742005061110830865800380706787109375;1.9784281704870083640201983143924735486507415771484375;-1.20241292265631471991582657210528850555419921875;-1.683027281503317595934277051128447055816650390625;-1.3268256885653764154398004393442533910274505615234375;-0.467202654118490323664758534505381248891353607177734375]
      mask Display: e = 0.06;c1 = [120 150 230]/255;c2 = ([120 150 230]+0)/383;c3 = ([120 150 230]+128)/383;patch([0 1 1 0],[0 0 1 1],c1);patch([0 1 1 1-e 1-e 0+e],[0 0 1 1-e 0+e 0+e],c2);patch([0 0 1 1-e 0+e 0+e],[0 1 1 1-e 1-e 0+e],c3);plot([0 1 1 0 0],[0 0 1 1 0]);disp('Weights');
  "IW{1,1}(218,:)'" : Constant  Value=[1.62674621779018213629797173780389130115509033203125;-1.5297314255324836462790472069173119962215423583984375;-1.813368031825123072309224880882538855075836181640625;0.55217857691856997437440668363706208765506744384765625;1.9026548993400707043832653653225861489772796630859375;-0.10371092739508745717014193132854416035115718841552734375]
      mask Display: e = 0.06;c1 = [120 150 230]/255;c2 = ([120 150 230]+0)/383;c3 = ([120 150 230]+128)/383;patch([0 1 1 0],[0 0 1 1],c1);patch([0 1 1 1-e 1-e 0+e],[0 0 1 1-e 0+e 0+e],c2);patch([0 0 1 1-e 0+e 0+e],[0 1 1 1-e 1-e 0+e],c3);plot([0 1 1 0 0],[0 0 1 1 0]);disp('Weights');
  "IW{1,1}(219,:)'" : Constant  Value=[-1.3157615374295132948390119054238311946392059326171875;0.08825968909064400846897768815324525348842144012451171875;1.63927264441782227777366642840206623077392578125;1.444051965706982354475940155680291354656219482421875;-1.647806619289605034595069810166023671627044677734375;1.657214308830301074948465611669234931468963623046875]
      mask Display: e = 0.06;c1 = [120 150 230]/255;c2 = ([120 150 230]+0)/383;c3 = ([120 150 230]+128)/383;patch([0 1 1 0],[0 0 1 1],c1);patch([0 1 1 1-e 1-e 0+e],[0 0 1 1-e 0+e 0+e],c2);patch([0 0 1 1-e 0+e 0+e],[0 1 1 1-e 1-e 0+e],c3);plot([0 1 1 0 0],[0 0 1 1 0]);disp('Weights');
  "IW{1,1}(22,:)'" : Constant  Value=[0.63771519115577757208512821307522244751453399658203125;-1.1559336052855042620279846232733689248561859130859375;1.715934070695071422818500650464557111263275146484375;2.423566713433178865244599364814348518848419189453125;0.3707885456800956713863115510321222245693206787109375;1.2289902227776756671318025837535969913005828857421875]
      mask Display: e = 0.06;c1 = [120 150 230]/255;c2 = ([120 150 230]+0)/383;c3 = ([120 150 230]+128)/383;patch([0 1 1 0],[0 0 1 1],c1);patch([0 1 1 1-e 1-e 0+e],[0 0 1 1-e 0+e 0+e],c2);patch([0 0 1 1-e 0+e 0+e],[0 1 1 1-e 1-e 0+e],c3);plot([0 1 1 0 0],[0 0 1 1 0]);disp('Weights');
  "IW{1,1}(220,:)'" : Constant  Value=[0.62632170272002041233605496017844416201114654541015625;-0.425819563886678020825371504542999900877475738525390625;1.6484321075406345169511723725008778274059295654296875;0.9475430874532067004878399529843591153621673583984375;2.539580071729802046576196516980417072772979736328125;1.2707158111801302169396876706741750240325927734375]
      mask Display: e = 0.06;c1 = [120 150 230]/255;c2 = ([120 150 230]+0)/383;c3 = ([120 150 230]+128)/383;patch([0 1 1 0],[0 0 1 1],c1);patch([0 1 1 1-e 1-e 0+e],[0 0 1 1-e 0+e 0+e],c2);patch([0 0 1 1-e 0+e 0+e],[0 1 1 1-e 1-e 0+e],c3);plot([0 1 1 0 0],[0 0 1 1 0]);disp('Weights');
  "IW{1,1}(221,:)'" : Constant  Value=[1.7247629364909256022286854204139672219753265380859375;-1.663463512806109267927467953995801508426666259765625;-1.6261937767632854701105316053144633769989013671875;1.36463774735300180651620394201017916202545166015625;1.0236130261641920302650987650849856436252593994140625;0.99980523174541569009221575470292009413242340087890625]
      mask Display: e = 0.06;c1 = [120 150 230]/255;c2 = ([120 150 230]+0)/383;c3 = ([120 150 230]+128)/383;patch([0 1 1 0],[0 0 1 1],c1);patch([0 1 1 1-e 1-e 0+e],[0 0 1 1-e 0+e 0+e],c2);patch([0 0 1 1-e 0+e 0+e],[0 1 1 1-e 1-e 0+e],c3);plot([0 1 1 0 0],[0 0 1 1 0]);disp('Weights');
  "IW{1,1}(222,:)'" : Constant  Value=[-1.2935853032058564071604678247240372002124786376953125;-0.141089521966903941319060322712175548076629638671875;-1.0333188079808925952107756529585458338260650634765625;1.7205760322900924830236135676386766135692596435546875;-0.7476959870354977777395788507419638335704803466796875;2.082681383030383859278344971244223415851593017578125]
      mask Display: e = 0.06;c1 = [120 150 230]/255;c2 = ([120 150 230]+0)/383;c3 = ([120 150 230]+128)/383;patch([0 1 1 0],[0 0 1 1],c1);patch([0 1 1 1-e 1-e 0+e],[0 0 1 1-e 0+e 0+e],c2);patch([0 0 1 1-e 0+e 0+e],[0 1 1 1-e 1-e 0+e],c3);plot([0 1 1 0 0],[0 0 1 1 0]);disp('Weights');
  "IW{1,1}(223,:)'" : Constant  Value=[1.713424278934555733400202370830811560153961181640625;-0.8687226502849352272050964529626071453094482421875;0.38487458106518579459276452325866557657718658447265625;-1.7240131023806328780523244859068654477596282958984375;1.6569765301512651145543486563838087022304534912109375;1.6536402295346501745143541484139859676361083984375]
      mask Display: e = 0.06;c1 = [120 150 230]/255;c2 = ([120 150 230]+0)/383;c3 = ([120 150 230]+128)/383;patch([0 1 1 0],[0 0 1 1],c1);patch([0 1 1 1-e 1-e 0+e],[0 0 1 1-e 0+e 0+e],c2);patch([0 0 1 1-e 0+e 0+e],[0 1 1 1-e 1-e 0+e],c3);plot([0 1 1 0 0],[0 0 1 1 0]);disp('Weights');
  "IW{1,1}(224,:)'" : Constant  Value=[-0.314723904299519297023124408951844088733196258544921875;2.4154226166680121679064541240222752094268798828125;0.8396950902435149632907496197731234133243560791015625;1.2845829904335082094490871895686723291873931884765625;-0.7454697859934833470418880096985958516597747802734375;-1.6882906523307268376044021351845003664493560791015625]
      mask Display: e = 0.06;c1 = [120 150 230]/255;c2 = ([120 150 230]+0)/383;c3 = ([120 150 230]+128)/383;patch([0 1 1 0],[0 0 1 1],c1);patch([0 1 1 1-e 1-e 0+e],[0 0 1 1-e 0+e 0+e],c2);patch([0 0 1 1-e 0+e 0+e],[0 1 1 1-e 1-e 0+e],c3);plot([0 1 1 0 0],[0 0 1 1 0]);disp('Weights');
  "IW{1,1}(225,:)'" : Constant  Value=[-1.199526573694594144825487092020921409130096435546875;-1.5870437011611067124050578058813698589801788330078125;-1.67695881983522188107826877967454493045806884765625;1.52586362920298057588297524489462375640869140625;0.01961121429502536706035442648499156348407268524169921875;-1.7580425632548088987761047974345274269580841064453125]
      mask Display: e = 0.06;c1 = [120 150 230]/255;c2 = ([120 150 230]+0)/383;c3 = ([120 150 230]+128)/383;patch([0 1 1 0],[0 0 1 1],c1);patch([0 1 1 1-e 1-e 0+e],[0 0 1 1-e 0+e 0+e],c2);patch([0 0 1 1-e 0+e 0+e],[0 1 1 1-e 1-e 0+e],c3);plot([0 1 1 0 0],[0 0 1 1 0]);disp('Weights');
  "IW{1,1}(226,:)'" : Constant  Value=[-1.4456591001983725153223758752574212849140167236328125;0.82982417706686317782072137561044655740261077880859375;-1.1532850882815528503755331257707439363002777099609375;-0.5305843095757865057748858816921710968017578125;1.9793436991090309629015564496512524783611297607421875;1.8110201172705060468359761216561309993267059326171875]
      mask Display: e = 0.06;c1 = [120 150 230]/255;c2 = ([120 150 230]+0)/383;c3 = ([120 150 230]+128)/383;patch([0 1 1 0],[0 0 1 1],c1);patch([0 1 1 1-e 1-e 0+e],[0 0 1 1-e 0+e 0+e],c2);patch([0 0 1 1-e 0+e 0+e],[0 1 1 1-e 1-e 0+e],c3);plot([0 1 1 0 0],[0 0 1 1 0]);disp('Weights');
  "IW{1,1}(227,:)'" : Constant  Value=[1.014731025965392330334680082160048186779022216796875;0.7023474349388101334312750623212195932865142822265625;-1.6623376999899386330383777021779678761959075927734375;-0.05054911212968084266439205975984805263578891754150390625;1.944899105513986370397105929441750049591064453125;-2.0557537945897639275472101871855556964874267578125]
      mask Display: e = 0.06;c1 = [120 150 230]/255;c2 = ([120 150 230]+0)/383;c3 = ([120 150 230]+128)/383;patch([0 1 1 0],[0 0 1 1],c1);patch([0 1 1 1-e 1-e 0+e],[0 0 1 1-e 0+e 0+e],c2);patch([0 0 1 1-e 0+e 0+e],[0 1 1 1-e 1-e 0+e],c3);plot([0 1 1 0 0],[0 0 1 1 0]);disp('Weights');
  "IW{1,1}(228,:)'" : Constant  Value=[1.4555069704306629052581456562620587646961212158203125;-1.68092481352275679995500468066893517971038818359375;1.375501288925146337049909561756066977977752685546875;-1.0657153359500812772608924205997027456760406494140625;-0.842059929107076055032621297868900001049041748046875;1.4106459917389175817703517168411053717136383056640625]
      mask Display: e = 0.06;c1 = [120 150 230]/255;c2 = ([120 150 230]+0)/383;c3 = ([120 150 230]+128)/383;patch([0 1 1 0],[0 0 1 1],c1);patch([0 1 1 1-e 1-e 0+e],[0 0 1 1-e 0+e 0+e],c2);patch([0 0 1 1-e 0+e 0+e],[0 1 1 1-e 1-e 0+e],c3);plot([0 1 1 0 0],[0 0 1 1 0]);disp('Weights');
  "IW{1,1}(229,:)'" : Constant  Value=[1.204967323373444809675447686458937823772430419921875;1.662567310708471968183630451676435768604278564453125;0.3086626702693167079161185029079206287860870361328125;1.270608334462326016733868527808226644992828369140625;1.43942555734938171241310556069947779178619384765625;2.031504475629501538236354463151656091213226318359375]
      mask Display: e = 0.06;c1 = [120 150 230]/255;c2 = ([120 150 230]+0)/383;c3 = ([120 150 230]+128)/383;patch([0 1 1 0],[0 0 1 1],c1);patch([0 1 1 1-e 1-e 0+e],[0 0 1 1-e 0+e 0+e],c2);patch([0 0 1 1-e 0+e 0+e],[0 1 1 1-e 1-e 0+e],c3);plot([0 1 1 0 0],[0 0 1 1 0]);disp('Weights');
  "IW{1,1}(23,:)'" : Constant  Value=[0.31959439140702083914646891571464948356151580810546875;-0.7525022009717530213634972824365831911563873291015625;0.47180578565993702699898904029396362602710723876953125;0.40770114175949656587505387506098486483097076416015625;-0.5473071764532446703555024214438162744045257568359375;-3.332830178229623907526502080145291984081268310546875]
      mask Display: e = 0.06;c1 = [120 150 230]/255;c2 = ([120 150 230]+0)/383;c3 = ([120 150 230]+128)/383;patch([0 1 1 0],[0 0 1 1],c1);patch([0 1 1 1-e 1-e 0+e],[0 0 1 1-e 0+e 0+e],c2);patch([0 0 1 1-e 0+e 0+e],[0 1 1 1-e 1-e 0+e],c3);plot([0 1 1 0 0],[0 0 1 1 0]);disp('Weights');
  "IW{1,1}(230,:)'" : Constant  Value=[-1.1726321162715167556456208330928348004817962646484375;2.267480251390911138997807938721962273120880126953125;-1.394305902030911425981685169972479343414306640625;-0.441302491964828347281724063577712513506412506103515625;1.26860735055962781103744418942369520664215087890625;1.665325688051369379394373027025721967220306396484375]
      mask Display: e = 0.06;c1 = [120 150 230]/255;c2 = ([120 150 230]+0)/383;c3 = ([120 150 230]+128)/383;patch([0 1 1 0],[0 0 1 1],c1);patch([0 1 1 1-e 1-e 0+e],[0 0 1 1-e 0+e 0+e],c2);patch([0 0 1 1-e 0+e 0+e],[0 1 1 1-e 1-e 0+e],c3);plot([0 1 1 0 0],[0 0 1 1 0]);disp('Weights');
  "IW{1,1}(231,:)'" : Constant  Value=[2.132335156156559552442786298342980444431304931640625;0.801268195218023837611553972237743437290191650390625;0.73362478561277544297780650595086626708507537841796875;2.33803937734892830491162385442294180393218994140625;0.80790450286838810800560395364300347864627838134765625;0.959649357428248972468054489581845700740814208984375]
      mask Display: e = 0.06;c1 = [120 150 230]/255;c2 = ([120 150 230]+0)/383;c3 = ([120 150 230]+128)/383;patch([0 1 1 0],[0 0 1 1],c1);patch([0 1 1 1-e 1-e 0+e],[0 0 1 1-e 0+e 0+e],c2);patch([0 0 1 1-e 0+e 0+e],[0 1 1 1-e 1-e 0+e],c3);plot([0 1 1 0 0],[0 0 1 1 0]);disp('Weights');
  "IW{1,1}(232,:)'" : Constant  Value=[-2.029729851321800282448748475871980190277099609375;1.6441431484411046515248244759277440607547760009765625;-1.7524310512531602324060031605768017470836639404296875;0.5197891934195786323158472441718913614749908447265625;-0.6771598821366868747873013489879667758941650390625;0.73478102164523095840564792524673976004123687744140625]
      mask Display: e = 0.06;c1 = [120 150 230]/255;c2 = ([120 150 230]+0)/383;c3 = ([120 150 230]+128)/383;patch([0 1 1 0],[0 0 1 1],c1);patch([0 1 1 1-e 1-e 0+e],[0 0 1 1-e 0+e 0+e],c2);patch([0 0 1 1-e 0+e 0+e],[0 1 1 1-e 1-e 0+e],c3);plot([0 1 1 0 0],[0 0 1 1 0]);disp('Weights');
  "IW{1,1}(233,:)'" : Constant  Value=[-0.8040279656835520594171384800574742257595062255859375;0.7740774784149329068583256230340339243412017822265625;-2.556123543353735261263182110269553959369659423828125;-0.76470715437029379568656395349535159766674041748046875;-1.76751182117990968123422135249711573123931884765625;-0.4985691948945600859843807484139688313007354736328125]
      mask Display: e = 0.06;c1 = [120 150 230]/255;c2 = ([120 150 230]+0)/383;c3 = ([120 150 230]+128)/383;patch([0 1 1 0],[0 0 1 1],c1);patch([0 1 1 1-e 1-e 0+e],[0 0 1 1-e 0+e 0+e],c2);patch([0 0 1 1-e 0+e 0+e],[0 1 1 1-e 1-e 0+e],c3);plot([0 1 1 0 0],[0 0 1 1 0]);disp('Weights');
  "IW{1,1}(234,:)'" : Constant  Value=[0.88142215738313023365435583400540053844451904296875;2.29719569008626667283579081413336098194122314453125;0.2023511561317128393255870832945220172405242919921875;-1.3202628854041080774806005138088949024677276611328125;-2.01687475470131882815394419594667851924896240234375;-0.759985148936209053971424509654752910137176513671875]
      mask Display: e = 0.06;c1 = [120 150 230]/255;c2 = ([120 150 230]+0)/383;c3 = ([120 150 230]+128)/383;patch([0 1 1 0],[0 0 1 1],c1);patch([0 1 1 1-e 1-e 0+e],[0 0 1 1-e 0+e 0+e],c2);patch([0 0 1 1-e 0+e 0+e],[0 1 1 1-e 1-e 0+e],c3);plot([0 1 1 0 0],[0 0 1 1 0]);disp('Weights');
  "IW{1,1}(235,:)'" : Constant  Value=[-1.6834471536882846809390912312665022909641265869140625;0.9900656020110798483102598765981383621692657470703125;-0.6377971221194231876694402672001160681247711181640625;-1.7512715234246767348480489090434275567531585693359375;-1.014625650114747923424829423311166465282440185546875;-1.842350786026698106212506900192238390445709228515625]
      mask Display: e = 0.06;c1 = [120 150 230]/255;c2 = ([120 150 230]+0)/383;c3 = ([120 150 230]+128)/383;patch([0 1 1 0],[0 0 1 1],c1);patch([0 1 1 1-e 1-e 0+e],[0 0 1 1-e 0+e 0+e],c2);patch([0 0 1 1-e 0+e 0+e],[0 1 1 1-e 1-e 0+e],c3);plot([0 1 1 0 0],[0 0 1 1 0]);disp('Weights');
  "IW{1,1}(236,:)'" : Constant  Value=[-2.13592806606213780895586751285009086132049560546875;-2.20140823764449322652581031434237957000732421875;-0.327714061396291056471596903065801598131656646728515625;0.3796283170156244946014112429111264646053314208984375;-1.5278179042640733786839746244368143379688262939453125;-0.70726056691212890736863982965587638318538665771484375]
      mask Display: e = 0.06;c1 = [120 150 230]/255;c2 = ([120 150 230]+0)/383;c3 = ([120 150 230]+128)/383;patch([0 1 1 0],[0 0 1 1],c1);patch([0 1 1 1-e 1-e 0+e],[0 0 1 1-e 0+e 0+e],c2);patch([0 0 1 1-e 0+e 0+e],[0 1 1 1-e 1-e 0+e],c3);plot([0 1 1 0 0],[0 0 1 1 0]);disp('Weights');
  "IW{1,1}(237,:)'" : Constant  Value=[0.264961354768516177404791278604534454643726348876953125;-2.136602668481032640812600220669992268085479736328125;-1.1096440473080024791130426820018328726291656494140625;-0.74546619354720655703516740686609409749507904052734375;-1.0469593235608651848878025703015737235546112060546875;1.5169739009134473040063539883703924715518951416015625]
      mask Display: e = 0.06;c1 = [120 150 230]/255;c2 = ([120 150 230]+0)/383;c3 = ([120 150 230]+128)/383;patch([0 1 1 0],[0 0 1 1],c1);patch([0 1 1 1-e 1-e 0+e],[0 0 1 1-e 0+e 0+e],c2);patch([0 0 1 1-e 0+e 0+e],[0 1 1 1-e 1-e 0+e],c3);plot([0 1 1 0 0],[0 0 1 1 0]);disp('Weights');
  "IW{1,1}(238,:)'" : Constant  Value=[0.68372357841331832251086098040104843676090240478515625;1.580004886198192348700786169501952826976776123046875;-0.1813752287556803233226077054496272467076778411865234375;0.491560057163365315968661661827354691922664642333984375;2.20515138613043593096563199651427567005157470703125;-2.287347244742514273951883296831510961055755615234375]
      mask Display: e = 0.06;c1 = [120 150 230]/255;c2 = ([120 150 230]+0)/383;c3 = ([120 150 230]+128)/383;patch([0 1 1 0],[0 0 1 1],c1);patch([0 1 1 1-e 1-e 0+e],[0 0 1 1-e 0+e 0+e],c2);patch([0 0 1 1-e 0+e 0+e],[0 1 1 1-e 1-e 0+e],c3);plot([0 1 1 0 0],[0 0 1 1 0]);disp('Weights');
  "IW{1,1}(239,:)'" : Constant  Value=[-1.3007777455384121889636617197538726031780242919921875;-0.7481164586763657808887728606350719928741455078125;-1.24249602441393580676276542362757027149200439453125;-2.407212089299964219435423729009926319122314453125;0.46290992633993754967747236150898970663547515869140625;-1.853633671677172412017853275756351649761199951171875]
      mask Display: e = 0.06;c1 = [120 150 230]/255;c2 = ([120 150 230]+0)/383;c3 = ([120 150 230]+128)/383;patch([0 1 1 0],[0 0 1 1],c1);patch([0 1 1 1-e 1-e 0+e],[0 0 1 1-e 0+e 0+e],c2);patch([0 0 1 1-e 0+e 0+e],[0 1 1 1-e 1-e 0+e],c3);plot([0 1 1 0 0],[0 0 1 1 0]);disp('Weights');
  "IW{1,1}(24,:)'" : Constant  Value=[0.414534511194227184294192056768224574625492095947265625;-0.078843509887748630671211458320613019168376922607421875;1.17723874363055802660937843029387295246124267578125;1.899084867954731858930017551756463944911956787109375;-2.056062821165285381397325181751511991024017333984375;1.65347833109458530742585935513488948345184326171875]
      mask Display: e = 0.06;c1 = [120 150 230]/255;c2 = ([120 150 230]+0)/383;c3 = ([120 150 230]+128)/383;patch([0 1 1 0],[0 0 1 1],c1);patch([0 1 1 1-e 1-e 0+e],[0 0 1 1-e 0+e 0+e],c2);patch([0 0 1 1-e 0+e 0+e],[0 1 1 1-e 1-e 0+e],c3);plot([0 1 1 0 0],[0 0 1 1 0]);disp('Weights');
  "IW{1,1}(240,:)'" : Constant  Value=[0.64743264701626646040466539488988928496837615966796875;-0.99129246170208051847083652319270186126232147216796875;-2.330743832851787100679530340130440890789031982421875;1.7155561180544316446372477003023959696292877197265625;0.26629597716655484251901953030028380453586578369140625;-0.99169302058436337166114071806077845394611358642578125]
      mask Display: e = 0.06;c1 = [120 150 230]/255;c2 = ([120 150 230]+0)/383;c3 = ([120 150 230]+128)/383;patch([0 1 1 0],[0 0 1 1],c1);patch([0 1 1 1-e 1-e 0+e],[0 0 1 1-e 0+e 0+e],c2);patch([0 0 1 1-e 0+e 0+e],[0 1 1 1-e 1-e 0+e],c3);plot([0 1 1 0 0],[0 0 1 1 0]);disp('Weights');
  "IW{1,1}(241,:)'" : Constant  Value=[0.147280406808535158091899575083516538143157958984375;-1.7279854044196933937627136401715688407421112060546875;1.928166548588996054292010740027762949466705322265625;-1.4460925847444647818207386080757714807987213134765625;-1.154414598839850203404466810752637684345245361328125;1.4528991481366821947318612728849984705448150634765625]
      mask Display: e = 0.06;c1 = [120 150 230]/255;c2 = ([120 150 230]+0)/383;c3 = ([120 150 230]+128)/383;patch([0 1 1 0],[0 0 1 1],c1);patch([0 1 1 1-e 1-e 0+e],[0 0 1 1-e 0+e 0+e],c2);patch([0 0 1 1-e 0+e 0+e],[0 1 1 1-e 1-e 0+e],c3);plot([0 1 1 0 0],[0 0 1 1 0]);disp('Weights');
  "IW{1,1}(242,:)'" : Constant  Value=[0.05569561416268985210020758813698193989694118499755859375;-2.174407578531912577091134153306484222412109375;-0.053317784151465201503139468286462943069636821746826171875;1.7342513859550516830410060720168985426425933837890625;1.9408721298394893128858029740513302385807037353515625;0.275896543337406818796608831689809449017047882080078125]
      mask Display: e = 0.06;c1 = [120 150 230]/255;c2 = ([120 150 230]+0)/383;c3 = ([120 150 230]+128)/383;patch([0 1 1 0],[0 0 1 1],c1);patch([0 1 1 1-e 1-e 0+e],[0 0 1 1-e 0+e 0+e],c2);patch([0 0 1 1-e 0+e 0+e],[0 1 1 1-e 1-e 0+e],c3);plot([0 1 1 0 0],[0 0 1 1 0]);disp('Weights');
  "IW{1,1}(243,:)'" : Constant  Value=[1.0901118503631159750710821754182688891887664794921875;-0.2392981799300385181705763670834130607545375823974609375;-1.1572574849862038437464661910780705511569976806640625;-1.44902860602228233943833402008749544620513916015625;-2.34853245026754553492764898692257702350616455078125;-0.80630256705197445032951009125099517405033111572265625]
      mask Display: e = 0.06;c1 = [120 150 230]/255;c2 = ([120 150 230]+0)/383;c3 = ([120 150 230]+128)/383;patch([0 1 1 0],[0 0 1 1],c1);patch([0 1 1 1-e 1-e 0+e],[0 0 1 1-e 0+e 0+e],c2);patch([0 0 1 1-e 0+e 0+e],[0 1 1 1-e 1-e 0+e],c3);plot([0 1 1 0 0],[0 0 1 1 0]);disp('Weights');
  "IW{1,1}(244,:)'" : Constant  Value=[-0.564618296368989636135893306345678865909576416015625;1.658137711451836526777015023981221020221710205078125;1.80363868213402778195586506626568734645843505859375;-0.11585097506638518394250780829679570160806179046630859375;-1.6692483102404158668008449240005575120449066162109375;1.274777359352641692424867869704030454158782958984375]
      mask Display: e = 0.06;c1 = [120 150 230]/255;c2 = ([120 150 230]+0)/383;c3 = ([120 150 230]+128)/383;patch([0 1 1 0],[0 0 1 1],c1);patch([0 1 1 1-e 1-e 0+e],[0 0 1 1-e 0+e 0+e],c2);patch([0 0 1 1-e 0+e 0+e],[0 1 1 1-e 1-e 0+e],c3);plot([0 1 1 0 0],[0 0 1 1 0]);disp('Weights');
  "IW{1,1}(245,:)'" : Constant  Value=[0.60233977140735939226345863062306307256221771240234375;1.3774404586162212194011544852401129901409149169921875;-1.99147388028887828426150008453987538814544677734375;1.2691401150423009536183371892548166215419769287109375;0.7538173055407406675243464633240364491939544677734375;1.986986769638458216746812468045391142368316650390625]
      mask Display: e = 0.06;c1 = [120 150 230]/255;c2 = ([120 150 230]+0)/383;c3 = ([120 150 230]+128)/383;patch([0 1 1 0],[0 0 1 1],c1);patch([0 1 1 1-e 1-e 0+e],[0 0 1 1-e 0+e 0+e],c2);patch([0 0 1 1-e 0+e 0+e],[0 1 1 1-e 1-e 0+e],c3);plot([0 1 1 0 0],[0 0 1 1 0]);disp('Weights');
  "IW{1,1}(246,:)'" : Constant  Value=[-1.1237513488300099329109116297331638634204864501953125;2.384016928810828606088989545241929590702056884765625;0.49433003417196508255671005827025510370731353759765625;0.2206044592875971155354619668287341482937335968017578125;2.0770736827848761407722122385166585445404052734375;0.374906706531195954568147499230690300464630126953125]
      mask Display: e = 0.06;c1 = [120 150 230]/255;c2 = ([120 150 230]+0)/383;c3 = ([120 150 230]+128)/383;patch([0 1 1 0],[0 0 1 1],c1);patch([0 1 1 1-e 1-e 0+e],[0 0 1 1-e 0+e 0+e],c2);patch([0 0 1 1-e 0+e 0+e],[0 1 1 1-e 1-e 0+e],c3);plot([0 1 1 0 0],[0 0 1 1 0]);disp('Weights');
  "IW{1,1}(247,:)'" : Constant  Value=[-2.461469833998963796517500668414868414402008056640625;1.3702579762036826149795842866296879947185516357421875;-2.023961055611118720065633169724605977535247802734375;0.76602711039308657436919247629703022539615631103515625;-0.65280103283954737936056744729285128414630889892578125;0.346269564921099892718103774313931353390216827392578125]
      mask Display: e = 0.06;c1 = [120 150 230]/255;c2 = ([120 150 230]+0)/383;c3 = ([120 150 230]+128)/383;patch([0 1 1 0],[0 0 1 1],c1);patch([0 1 1 1-e 1-e 0+e],[0 0 1 1-e 0+e 0+e],c2);patch([0 0 1 1-e 0+e 0+e],[0 1 1 1-e 1-e 0+e],c3);plot([0 1 1 0 0],[0 0 1 1 0]);disp('Weights');
  "IW{1,1}(248,:)'" : Constant  Value=[0.945951015333447831068269806564785540103912353515625;-1.0625231201944369541223522901418618857860565185546875;2.05249807510492932038914659642614424228668212890625;1.806817411646109317047148579149506986141204833984375;1.148322050981525510593428407446481287479400634765625;0.74197218605838577420996671207831241190433502197265625]
      mask Display: e = 0.06;c1 = [120 150 230]/255;c2 = ([120 150 230]+0)/383;c3 = ([120 150 230]+128)/383;patch([0 1 1 0],[0 0 1 1],c1);patch([0 1 1 1-e 1-e 0+e],[0 0 1 1-e 0+e 0+e],c2);patch([0 0 1 1-e 0+e 0+e],[0 1 1 1-e 1-e 0+e],c3);plot([0 1 1 0 0],[0 0 1 1 0]);disp('Weights');
  "IW{1,1}(249,:)'" : Constant  Value=[-1.8628008467116765611848450134857557713985443115234375;-0.05704778297077195414743755463859997689723968505859375;1.90832130451028181283845697180368006229400634765625;-1.14652574455370181993885125848464667797088623046875;1.5094757643240501732151415126281790435314178466796875;-0.54187679832525315060109960541012696921825408935546875]
      mask Display: e = 0.06;c1 = [120 150 230]/255;c2 = ([120 150 230]+0)/383;c3 = ([120 150 230]+128)/383;patch([0 1 1 0],[0 0 1 1],c1);patch([0 1 1 1-e 1-e 0+e],[0 0 1 1-e 0+e 0+e],c2);patch([0 0 1 1-e 0+e 0+e],[0 1 1 1-e 1-e 0+e],c3);plot([0 1 1 0 0],[0 0 1 1 0]);disp('Weights');
  "IW{1,1}(25,:)'" : Constant  Value=[-1.596595900351970964692327470402233302593231201171875;2.418019092355714771969132925732992589473724365234375;1.2427558360778447887895481471787206828594207763671875;-0.2349889807069429903396695635819924063980579376220703125;1.25019653280320763855115728802047669887542724609375;-0.10229557286418812511730180858648964203894138336181640625]
      mask Display: e = 0.06;c1 = [120 150 230]/255;c2 = ([120 150 230]+0)/383;c3 = ([120 150 230]+128)/383;patch([0 1 1 0],[0 0 1 1],c1);patch([0 1 1 1-e 1-e 0+e],[0 0 1 1-e 0+e 0+e],c2);patch([0 0 1 1-e 0+e 0+e],[0 1 1 1-e 1-e 0+e],c3);plot([0 1 1 0 0],[0 0 1 1 0]);disp('Weights');
  "IW{1,1}(250,:)'" : Constant  Value=[-0.703505186641293800420271509210579097270965576171875;1.1738008436211797569370673954836092889308929443359375;-0.047186018677918238617419177671763463877141475677490234375;0.75593253580854302686731216454063542187213897705078125;-2.278657884983470438555741566233336925506591796875;2.206923570952060043026676794397644698619842529296875]
      mask Display: e = 0.06;c1 = [120 150 230]/255;c2 = ([120 150 230]+0)/383;c3 = ([120 150 230]+128)/383;patch([0 1 1 0],[0 0 1 1],c1);patch([0 1 1 1-e 1-e 0+e],[0 0 1 1-e 0+e 0+e],c2);patch([0 0 1 1-e 0+e 0+e],[0 1 1 1-e 1-e 0+e],c3);plot([0 1 1 0 0],[0 0 1 1 0]);disp('Weights');
  "IW{1,1}(26,:)'" : Constant  Value=[0.0260399360515743104327324175528701744042336940765380859375;0.36843465276340736647142648507724516093730926513671875;2.563676686962169437578040742664597928524017333984375;-0.7884053035266254116919526495621539652347564697265625;0.59748773766266072282604682186502031981945037841796875;2.186779744096176703038736377493478357791900634765625]
      mask Display: e = 0.06;c1 = [120 150 230]/255;c2 = ([120 150 230]+0)/383;c3 = ([120 150 230]+128)/383;patch([0 1 1 0],[0 0 1 1],c1);patch([0 1 1 1-e 1-e 0+e],[0 0 1 1-e 0+e 0+e],c2);patch([0 0 1 1-e 0+e 0+e],[0 1 1 1-e 1-e 0+e],c3);plot([0 1 1 0 0],[0 0 1 1 0]);disp('Weights');
  "IW{1,1}(27,:)'" : Constant  Value=[-0.1611721191988953749696378281441866420209407806396484375;-0.49215069917449749681281900848262012004852294921875;1.60917214002707709141759551130235195159912109375;1.3030326022600597912770581388031132519245147705078125;-0.6144334636896535695171905899769626557826995849609375;-2.81996138135760165965848500491119921207427978515625]
      mask Display: e = 0.06;c1 = [120 150 230]/255;c2 = ([120 150 230]+0)/383;c3 = ([120 150 230]+128)/383;patch([0 1 1 0],[0 0 1 1],c1);patch([0 1 1 1-e 1-e 0+e],[0 0 1 1-e 0+e 0+e],c2);patch([0 0 1 1-e 0+e 0+e],[0 1 1 1-e 1-e 0+e],c3);plot([0 1 1 0 0],[0 0 1 1 0]);disp('Weights');
  "IW{1,1}(28,:)'" : Constant  Value=[2.59839262561484307667569737532176077365875244140625;-0.386512860509139521969501629428123123943805694580078125;0.60605616769667591814396701010991819202899932861328125;1.7292613632212248120367803494445979595184326171875;-0.4803725542046073382351778491283766925334930419921875;1.575469108264881956671388252289034426212310791015625]
      mask Display: e = 0.06;c1 = [120 150 230]/255;c2 = ([120 150 230]+0)/383;c3 = ([120 150 230]+128)/383;patch([0 1 1 0],[0 0 1 1],c1);patch([0 1 1 1-e 1-e 0+e],[0 0 1 1-e 0+e 0+e],c2);patch([0 0 1 1-e 0+e 0+e],[0 1 1 1-e 1-e 0+e],c3);plot([0 1 1 0 0],[0 0 1 1 0]);disp('Weights');
  "IW{1,1}(29,:)'" : Constant  Value=[0.340221210419808073321945585121284238994121551513671875;2.27667545478414101722819395945407450199127197265625;0.509882933711716557212412226363085210323333740234375;2.11231946756041022439376320107840001583099365234375;0.2151483437211192117910485421816702000796794891357421875;1.6220098949737522531222566612996160984039306640625]
      mask Display: e = 0.06;c1 = [120 150 230]/255;c2 = ([120 150 230]+0)/383;c3 = ([120 150 230]+128)/383;patch([0 1 1 0],[0 0 1 1],c1);patch([0 1 1 1-e 1-e 0+e],[0 0 1 1-e 0+e 0+e],c2);patch([0 0 1 1-e 0+e 0+e],[0 1 1 1-e 1-e 0+e],c3);plot([0 1 1 0 0],[0 0 1 1 0]);disp('Weights');
  "IW{1,1}(3,:)'" : Constant  Value=[2.11494965950875890570159754133783280849456787109375;-1.49889459822359416563131162547506392002105712890625;-1.4319744532759519639597556306398473680019378662109375;1.365928214336492363401021066238172352313995361328125;0.963395539943101564261951352818869054317474365234375;0.380398954592316707046251167412265203893184661865234375]
      mask Display: e = 0.06;c1 = [120 150 230]/255;c2 = ([120 150 230]+0)/383;c3 = ([120 150 230]+128)/383;patch([0 1 1 0],[0 0 1 1],c1);patch([0 1 1 1-e 1-e 0+e],[0 0 1 1-e 0+e 0+e],c2);patch([0 0 1 1-e 0+e 0+e],[0 1 1 1-e 1-e 0+e],c3);plot([0 1 1 0 0],[0 0 1 1 0]);disp('Weights');
  "IW{1,1}(30,:)'" : Constant  Value=[-1.7038555511492659011452133199782110750675201416015625;0.6869802477600093215670540303108282387256622314453125;0.1336493103584203978595468242929200641810894012451171875;-1.637876056727464391116200204123742878437042236328125;-2.180072714429866831409299265942536294460296630859375;0.458087101845869870686556168948300182819366455078125]
      mask Display: e = 0.06;c1 = [120 150 230]/255;c2 = ([120 150 230]+0)/383;c3 = ([120 150 230]+128)/383;patch([0 1 1 0],[0 0 1 1],c1);patch([0 1 1 1-e 1-e 0+e],[0 0 1 1-e 0+e 0+e],c2);patch([0 0 1 1-e 0+e 0+e],[0 1 1 1-e 1-e 0+e],c3);plot([0 1 1 0 0],[0 0 1 1 0]);disp('Weights');
  "IW{1,1}(31,:)'" : Constant  Value=[-1.727903060055431705421824517543427646160125732421875;-0.39132378442687698605340074209379963576793670654296875;2.21524972571179734615043344092555344104766845703125;1.686707033339410077843467661296017467975616455078125;-1.6104955629329691380036138070863671600818634033203125;0.0204272736335327186052435166629948071204125881195068359375]
      mask Display: e = 0.06;c1 = [120 150 230]/255;c2 = ([120 150 230]+0)/383;c3 = ([120 150 230]+128)/383;patch([0 1 1 0],[0 0 1 1],c1);patch([0 1 1 1-e 1-e 0+e],[0 0 1 1-e 0+e 0+e],c2);patch([0 0 1 1-e 0+e 0+e],[0 1 1 1-e 1-e 0+e],c3);plot([0 1 1 0 0],[0 0 1 1 0]);disp('Weights');
  "IW{1,1}(32,:)'" : Constant  Value=[1.286963512849421675809935550205409526824951171875;0.463824598267942922458217935854918323457241058349609375;-0.51188207832600973734571425666217692196369171142578125;-3.022792487633738200969446552335284650325775146484375;-0.77938696847050525917666163877584040164947509765625;0.267862923641156547294173151385621167719364166259765625]
      mask Display: e = 0.06;c1 = [120 150 230]/255;c2 = ([120 150 230]+0)/383;c3 = ([120 150 230]+128)/383;patch([0 1 1 0],[0 0 1 1],c1);patch([0 1 1 1-e 1-e 0+e],[0 0 1 1-e 0+e 0+e],c2);patch([0 0 1 1-e 0+e 0+e],[0 1 1 1-e 1-e 0+e],c3);plot([0 1 1 0 0],[0 0 1 1 0]);disp('Weights');
  "IW{1,1}(33,:)'" : Constant  Value=[-1.6284743339246021687216625650762580335140228271484375;1.9856671561060041941715326174744404852390289306640625;0.8031926609004360617660722709842957556247711181640625;1.350601304900914900741781821125186979770660400390625;-1.881004648742010232354004983790218830108642578125;-0.533249287037102615016692652716301381587982177734375]
      mask Display: e = 0.06;c1 = [120 150 230]/255;c2 = ([120 150 230]+0)/383;c3 = ([120 150 230]+128)/383;patch([0 1 1 0],[0 0 1 1],c1);patch([0 1 1 1-e 1-e 0+e],[0 0 1 1-e 0+e 0+e],c2);patch([0 0 1 1-e 0+e 0+e],[0 1 1 1-e 1-e 0+e],c3);plot([0 1 1 0 0],[0 0 1 1 0]);disp('Weights');
  "IW{1,1}(34,:)'" : Constant  Value=[-0.6970019961297311272829801964689977467060089111328125;1.503176910177999925366520983516238629817962646484375;-1.4527703832298612951490213163197040557861328125;-1.7987445822585332866339058455196209251880645751953125;2.317705294549423644667740518343634903430938720703125;0.283568928768719086264127327012829482555389404296875]
      mask Display: e = 0.06;c1 = [120 150 230]/255;c2 = ([120 150 230]+0)/383;c3 = ([120 150 230]+128)/383;patch([0 1 1 0],[0 0 1 1],c1);patch([0 1 1 1-e 1-e 0+e],[0 0 1 1-e 0+e 0+e],c2);patch([0 0 1 1-e 0+e 0+e],[0 1 1 1-e 1-e 0+e],c3);plot([0 1 1 0 0],[0 0 1 1 0]);disp('Weights');
  "IW{1,1}(35,:)'" : Constant  Value=[1.24849552706756572462154508684761822223663330078125;-2.094545195075002919082862717914395034313201904296875;1.364545971239798927143738183076493442058563232421875;-0.038075013109650467091338299496783292852342128753662109375;1.7744462558873816959703617612831294536590576171875;-1.1291436928395317540463338445988483726978302001953125]
      mask Display: e = 0.06;c1 = [120 150 230]/255;c2 = ([120 150 230]+0)/383;c3 = ([120 150 230]+128)/383;patch([0 1 1 0],[0 0 1 1],c1);patch([0 1 1 1-e 1-e 0+e],[0 0 1 1-e 0+e 0+e],c2);patch([0 0 1 1-e 0+e 0+e],[0 1 1 1-e 1-e 0+e],c3);plot([0 1 1 0 0],[0 0 1 1 0]);disp('Weights');
  "IW{1,1}(36,:)'" : Constant  Value=[0.7380863672114357232345582815469242632389068603515625;-0.5705865548557709221455525039345957338809967041015625;-1.5283855496886336045037069197860546410083770751953125;1.6113343561463768782715533234295435249805450439453125;1.9678522244506104765804366252268664538860321044921875;-1.6098709396589725439952189844916574656963348388671875]
      mask Display: e = 0.06;c1 = [120 150 230]/255;c2 = ([120 150 230]+0)/383;c3 = ([120 150 230]+128)/383;patch([0 1 1 0],[0 0 1 1],c1);patch([0 1 1 1-e 1-e 0+e],[0 0 1 1-e 0+e 0+e],c2);patch([0 0 1 1-e 0+e 0+e],[0 1 1 1-e 1-e 0+e],c3);plot([0 1 1 0 0],[0 0 1 1 0]);disp('Weights');
  "IW{1,1}(37,:)'" : Constant  Value=[-0.94596000111223943473959252514760009944438934326171875;1.4121569581011346183885279970127157866954803466796875;-1.746428824601853335707346559502184391021728515625;0.322474504119358906795156372027122415602207183837890625;1.748589160214093052303496733657084405422210693359375;1.9034231425666108261651743305264972150325775146484375]
      mask Display: e = 0.06;c1 = [120 150 230]/255;c2 = ([120 150 230]+0)/383;c3 = ([120 150 230]+128)/383;patch([0 1 1 0],[0 0 1 1],c1);patch([0 1 1 1-e 1-e 0+e],[0 0 1 1-e 0+e 0+e],c2);patch([0 0 1 1-e 0+e 0+e],[0 1 1 1-e 1-e 0+e],c3);plot([0 1 1 0 0],[0 0 1 1 0]);disp('Weights');
  "IW{1,1}(38,:)'" : Constant  Value=[1.627848175504742922470313715166412293910980224609375;-1.98001380858039954802052307059057056903839111328125;-1.2079168213032176470989043082226999104022979736328125;-1.23138610215121868662890847190283238887786865234375;-0.416697491509079032123707975188153795897960662841796875;-1.5462887339356559124325940501876175403594970703125]
      mask Display: e = 0.06;c1 = [120 150 230]/255;c2 = ([120 150 230]+0)/383;c3 = ([120 150 230]+128)/383;patch([0 1 1 0],[0 0 1 1],c1);patch([0 1 1 1-e 1-e 0+e],[0 0 1 1-e 0+e 0+e],c2);patch([0 0 1 1-e 0+e 0+e],[0 1 1 1-e 1-e 0+e],c3);plot([0 1 1 0 0],[0 0 1 1 0]);disp('Weights');
  "IW{1,1}(39,:)'" : Constant  Value=[-1.397668498137471626563410609378479421138763427734375;-1.6847903160257746701944370215642265975475311279296875;-1.776787984160506095321352404425852000713348388671875;-1.2311260069878040557256326792412437498569488525390625;-1.367893383191006062560290956753306090831756591796875;-0.6707716500970579698304163684952072799205780029296875]
      mask Display: e = 0.06;c1 = [120 150 230]/255;c2 = ([120 150 230]+0)/383;c3 = ([120 150 230]+128)/383;patch([0 1 1 0],[0 0 1 1],c1);patch([0 1 1 1-e 1-e 0+e],[0 0 1 1-e 0+e 0+e],c2);patch([0 0 1 1-e 0+e 0+e],[0 1 1 1-e 1-e 0+e],c3);plot([0 1 1 0 0],[0 0 1 1 0]);disp('Weights');
  "IW{1,1}(4,:)'" : Constant  Value=[-1.6932404554349533842838582131662406027317047119140625;0.8137165690186776156878067922662012279033660888671875;-1.153417449370521818963197802077047526836395263671875;-0.367374068370028117325176708618528209626674652099609375;1.9277237958806658912891407453571446239948272705078125;1.7793848197099924046682417611009441316127777099609375]
      mask Display: e = 0.06;c1 = [120 150 230]/255;c2 = ([120 150 230]+0)/383;c3 = ([120 150 230]+128)/383;patch([0 1 1 0],[0 0 1 1],c1);patch([0 1 1 1-e 1-e 0+e],[0 0 1 1-e 0+e 0+e],c2);patch([0 0 1 1-e 0+e 0+e],[0 1 1 1-e 1-e 0+e],c3);plot([0 1 1 0 0],[0 0 1 1 0]);disp('Weights');
  "IW{1,1}(40,:)'" : Constant  Value=[-1.9592625048109315599731417023576796054840087890625;-1.1576778564485257216887248432612977921962738037109375;-1.1744761449305751721539081700029782950878143310546875;0.124838254093939504674182217058842070400714874267578125;-2.060194654979061734678680295473895967006683349609375;-0.55041191325043481441525727859698235988616943359375]
      mask Display: e = 0.06;c1 = [120 150 230]/255;c2 = ([120 150 230]+0)/383;c3 = ([120 150 230]+128)/383;patch([0 1 1 0],[0 0 1 1],c1);patch([0 1 1 1-e 1-e 0+e],[0 0 1 1-e 0+e 0+e],c2);patch([0 0 1 1-e 0+e 0+e],[0 1 1 1-e 1-e 0+e],c3);plot([0 1 1 0 0],[0 0 1 1 0]);disp('Weights');
  "IW{1,1}(41,:)'" : Constant  Value=[0.8558277007060086649659069735207594931125640869140625;-2.008414960578638552846086895442567765712738037109375;-1.07065518470111076254625004366971552371978759765625;1.628799678311940279940017717308364808559417724609375;1.2566935093046629479118792005465365946292877197265625;1.5753260720696522501071967781172133982181549072265625]
      mask Display: e = 0.06;c1 = [120 150 230]/255;c2 = ([120 150 230]+0)/383;c3 = ([120 150 230]+128)/383;patch([0 1 1 0],[0 0 1 1],c1);patch([0 1 1 1-e 1-e 0+e],[0 0 1 1-e 0+e 0+e],c2);patch([0 0 1 1-e 0+e 0+e],[0 1 1 1-e 1-e 0+e],c3);plot([0 1 1 0 0],[0 0 1 1 0]);disp('Weights');
  "IW{1,1}(42,:)'" : Constant  Value=[1.2019239168726911781703847736935131251811981201171875;-1.41667280759498392939121913514100015163421630859375;2.36350510790793766346951088053174316883087158203125;-0.8688177627324993324009483330883085727691650390625;-0.6071184925851256242168574317474849522113800048828125;1.3838464408902988456162574948393739759922027587890625]
      mask Display: e = 0.06;c1 = [120 150 230]/255;c2 = ([120 150 230]+0)/383;c3 = ([120 150 230]+128)/383;patch([0 1 1 0],[0 0 1 1],c1);patch([0 1 1 1-e 1-e 0+e],[0 0 1 1-e 0+e 0+e],c2);patch([0 0 1 1-e 0+e 0+e],[0 1 1 1-e 1-e 0+e],c3);plot([0 1 1 0 0],[0 0 1 1 0]);disp('Weights');
  "IW{1,1}(43,:)'" : Constant  Value=[-1.9808662799750809124788020199048332870006561279296875;-0.0992316242280430749200803575149620883166790008544921875;0.474888546575503001090368115910678170621395111083984375;0.48705087149748427233220127163804136216640472412109375;-1.2494261297568005630864718114025890827178955078125;-2.054831995254450038856930405017919838428497314453125]
      mask Display: e = 0.06;c1 = [120 150 230]/255;c2 = ([120 150 230]+0)/383;c3 = ([120 150 230]+128)/383;patch([0 1 1 0],[0 0 1 1],c1);patch([0 1 1 1-e 1-e 0+e],[0 0 1 1-e 0+e 0+e],c2);patch([0 0 1 1-e 0+e 0+e],[0 1 1 1-e 1-e 0+e],c3);plot([0 1 1 0 0],[0 0 1 1 0]);disp('Weights');
  "IW{1,1}(44,:)'" : Constant  Value=[1.3787777149347835159431951979058794677257537841796875;1.371568115439391721821493774768896400928497314453125;-0.44089206769488609172213955389452166855335235595703125;-2.6632183519562016016379857319407165050506591796875;1.181963220510808820762349569122307002544403076171875;0.7347261199545653820308643844327889382839202880859375]
      mask Display: e = 0.06;c1 = [120 150 230]/255;c2 = ([120 150 230]+0)/383;c3 = ([120 150 230]+128)/383;patch([0 1 1 0],[0 0 1 1],c1);patch([0 1 1 1-e 1-e 0+e],[0 0 1 1-e 0+e 0+e],c2);patch([0 0 1 1-e 0+e 0+e],[0 1 1 1-e 1-e 0+e],c3);plot([0 1 1 0 0],[0 0 1 1 0]);disp('Weights');
  "IW{1,1}(45,:)'" : Constant  Value=[-2.377253094057432125651985188596881926059722900390625;-0.1740409848072168863541975269981776364147663116455078125;-1.3348469317542670520282399593270383775234222412109375;1.3223970864340877096054782668943516910076141357421875;-1.5821249558997190209908012548112310469150543212890625;-0.44219852888483490715998414088971912860870361328125]
      mask Display: e = 0.06;c1 = [120 150 230]/255;c2 = ([120 150 230]+0)/383;c3 = ([120 150 230]+128)/383;patch([0 1 1 0],[0 0 1 1],c1);patch([0 1 1 1-e 1-e 0+e],[0 0 1 1-e 0+e 0+e],c2);patch([0 0 1 1-e 0+e 0+e],[0 1 1 1-e 1-e 0+e],c3);plot([0 1 1 0 0],[0 0 1 1 0]);disp('Weights');
  "IW{1,1}(46,:)'" : Constant  Value=[1.1930146369796688077258295379579067230224609375;-1.2275965018079058044264684212976135313510894775390625;1.802264687519926855685525879380293190479278564453125;-0.91945694418180234919191207154653966426849365234375;-1.53130719969294659676961600780487060546875;-1.4323773469930973778474481150624342262744903564453125]
      mask Display: e = 0.06;c1 = [120 150 230]/255;c2 = ([120 150 230]+0)/383;c3 = ([120 150 230]+128)/383;patch([0 1 1 0],[0 0 1 1],c1);patch([0 1 1 1-e 1-e 0+e],[0 0 1 1-e 0+e 0+e],c2);patch([0 0 1 1-e 0+e 0+e],[0 1 1 1-e 1-e 0+e],c3);plot([0 1 1 0 0],[0 0 1 1 0]);disp('Weights');
  "IW{1,1}(47,:)'" : Constant  Value=[2.243010443370045958744185554678551852703094482421875;1.51469624390013368753216127515770494937896728515625;1.1216934013971260331032908652559854090213775634765625;0.313266893464598739083015743744908832013607025146484375;1.9655054051185325558748218099935911595821380615234375;-0.456830492117279163277743236903916113078594207763671875]
      mask Display: e = 0.06;c1 = [120 150 230]/255;c2 = ([120 150 230]+0)/383;c3 = ([120 150 230]+128)/383;patch([0 1 1 0],[0 0 1 1],c1);patch([0 1 1 1-e 1-e 0+e],[0 0 1 1-e 0+e 0+e],c2);patch([0 0 1 1-e 0+e 0+e],[0 1 1 1-e 1-e 0+e],c3);plot([0 1 1 0 0],[0 0 1 1 0]);disp('Weights');
  "IW{1,1}(48,:)'" : Constant  Value=[0.381932713027171910624701922642998397350311279296875;-2.44517636971219332053806283511221408843994140625;1.149981019683462779568117184680886566638946533203125;0.54017109849485700490134831852628849446773529052734375;2.020009678141807096807269772398285567760467529296875;-0.416340163757782877329560733414837159216403961181640625]
      mask Display: e = 0.06;c1 = [120 150 230]/255;c2 = ([120 150 230]+0)/383;c3 = ([120 150 230]+128)/383;patch([0 1 1 0],[0 0 1 1],c1);patch([0 1 1 1-e 1-e 0+e],[0 0 1 1-e 0+e 0+e],c2);patch([0 0 1 1-e 0+e 0+e],[0 1 1 1-e 1-e 0+e],c3);plot([0 1 1 0 0],[0 0 1 1 0]);disp('Weights');
  "IW{1,1}(49,:)'" : Constant  Value=[1.3192669689753777628737907434697262942790985107421875;-1.5005088552028624793166500239749439060688018798828125;-1.3090572062076548665032760254689492285251617431640625;-1.20816096904731917760500436997972428798675537109375;1.494538550341876881333291748887859284877777099609375;1.6043911915321587002836167812347412109375]
      mask Display: e = 0.06;c1 = [120 150 230]/255;c2 = ([120 150 230]+0)/383;c3 = ([120 150 230]+128)/383;patch([0 1 1 0],[0 0 1 1],c1);patch([0 1 1 1-e 1-e 0+e],[0 0 1 1-e 0+e 0+e],c2);patch([0 0 1 1-e 0+e 0+e],[0 1 1 1-e 1-e 0+e],c3);plot([0 1 1 0 0],[0 0 1 1 0]);disp('Weights');
  "IW{1,1}(5,:)'" : Constant  Value=[-0.98604862022325934223232479780563153326511383056640625;0.9213785085458006118841467468882910907268524169921875;-0.71990681313608462232878082431852817535400390625;1.6318798311312292526054079644381999969482421875;-2.36262983567610174162609837367199361324310302734375;1.5286546121831730005169447395019233226776123046875]
      mask Display: e = 0.06;c1 = [120 150 230]/255;c2 = ([120 150 230]+0)/383;c3 = ([120 150 230]+128)/383;patch([0 1 1 0],[0 0 1 1],c1);patch([0 1 1 1-e 1-e 0+e],[0 0 1 1-e 0+e 0+e],c2);patch([0 0 1 1-e 0+e 0+e],[0 1 1 1-e 1-e 0+e],c3);plot([0 1 1 0 0],[0 0 1 1 0]);disp('Weights');
  "IW{1,1}(50,:)'" : Constant  Value=[-1.9403086609293911379836572450585663318634033203125;1.771440594138320445694034788175486028194427490234375;-0.273340204551460297377474262248142622411251068115234375;-0.01407890546912314577721048181047081016004085540771484375;-1.8414695051257934377275660153827629983425140380859375;-1.400461011545559575353081527282483875751495361328125]
      mask Display: e = 0.06;c1 = [120 150 230]/255;c2 = ([120 150 230]+0)/383;c3 = ([120 150 230]+128)/383;patch([0 1 1 0],[0 0 1 1],c1);patch([0 1 1 1-e 1-e 0+e],[0 0 1 1-e 0+e 0+e],c2);patch([0 0 1 1-e 0+e 0+e],[0 1 1 1-e 1-e 0+e],c3);plot([0 1 1 0 0],[0 0 1 1 0]);disp('Weights');
  "IW{1,1}(51,:)'" : Constant  Value=[-1.24411345718127819282017298974096775054931640625;0.72382009839700833797593304552719928324222564697265625;1.357460292773067234151085358462296426296234130859375;1.696615707947863871396521062706597149372100830078125;-1.1828462391812870624363540628110058605670928955078125;2.02798451459934003793250667513348162174224853515625]
      mask Display: e = 0.06;c1 = [120 150 230]/255;c2 = ([120 150 230]+0)/383;c3 = ([120 150 230]+128)/383;patch([0 1 1 0],[0 0 1 1],c1);patch([0 1 1 1-e 1-e 0+e],[0 0 1 1-e 0+e 0+e],c2);patch([0 0 1 1-e 0+e 0+e],[0 1 1 1-e 1-e 0+e],c3);plot([0 1 1 0 0],[0 0 1 1 0]);disp('Weights');
  "IW{1,1}(52,:)'" : Constant  Value=[-2.186350758388125203879326363676227629184722900390625;0.06221246355607734646042672466137446463108062744140625;-2.009784285902932676748378071351908147335052490234375;-0.68890155163082500422433440689928829669952392578125;1.77271614262642085435572880669496953487396240234375;0.05701466379828827590880990783261950127780437469482421875]
      mask Display: e = 0.06;c1 = [120 150 230]/255;c2 = ([120 150 230]+0)/383;c3 = ([120 150 230]+128)/383;patch([0 1 1 0],[0 0 1 1],c1);patch([0 1 1 1-e 1-e 0+e],[0 0 1 1-e 0+e 0+e],c2);patch([0 0 1 1-e 0+e 0+e],[0 1 1 1-e 1-e 0+e],c3);plot([0 1 1 0 0],[0 0 1 1 0]);disp('Weights');
  "IW{1,1}(53,:)'" : Constant  Value=[1.0632930314392641246712400970864109694957733154296875;0.63856649930683329063896280786138959228992462158203125;1.3882905103576888006244871576200239360332489013671875;-2.06792102255520848785863563534803688526153564453125;1.4778077578546062742503863773890770971775054931640625;1.546509234395923026994523752364329993724822998046875]
      mask Display: e = 0.06;c1 = [120 150 230]/255;c2 = ([120 150 230]+0)/383;c3 = ([120 150 230]+128)/383;patch([0 1 1 0],[0 0 1 1],c1);patch([0 1 1 1-e 1-e 0+e],[0 0 1 1-e 0+e 0+e],c2);patch([0 0 1 1-e 0+e 0+e],[0 1 1 1-e 1-e 0+e],c3);plot([0 1 1 0 0],[0 0 1 1 0]);disp('Weights');
  "IW{1,1}(54,:)'" : Constant  Value=[-1.1109905686669476754246943528414703905582427978515625;1.6260081582830812063633629804826341569423675537109375;1.8971201902728556110133695256081409752368927001953125;0.52929512672506018322593490665894933044910430908203125;-1.3275396348580621452839523044531233608722686767578125;-1.695362855189987083548430746304802596569061279296875]
      mask Display: e = 0.06;c1 = [120 150 230]/255;c2 = ([120 150 230]+0)/383;c3 = ([120 150 230]+128)/383;patch([0 1 1 0],[0 0 1 1],c1);patch([0 1 1 1-e 1-e 0+e],[0 0 1 1-e 0+e 0+e],c2);patch([0 0 1 1-e 0+e 0+e],[0 1 1 1-e 1-e 0+e],c3);plot([0 1 1 0 0],[0 0 1 1 0]);disp('Weights');
  "IW{1,1}(55,:)'" : Constant  Value=[1.0783867935359332523859166030888445675373077392578125;-2.030960514507080372226255349232815206050872802734375;-1.6086075068077285710188562006806023418903350830078125;-1.2658296039810339461695321006118319928646087646484375;-0.79953185545210392337622806735453195869922637939453125;-1.19428331615911442753485971479676663875579833984375]
      mask Display: e = 0.06;c1 = [120 150 230]/255;c2 = ([120 150 230]+0)/383;c3 = ([120 150 230]+128)/383;patch([0 1 1 0],[0 0 1 1],c1);patch([0 1 1 1-e 1-e 0+e],[0 0 1 1-e 0+e 0+e],c2);patch([0 0 1 1-e 0+e 0+e],[0 1 1 1-e 1-e 0+e],c3);plot([0 1 1 0 0],[0 0 1 1 0]);disp('Weights');
  "IW{1,1}(56,:)'" : Constant  Value=[-0.03239004616421932436498565266447258181869983673095703125;-0.06853008536777606407586205250481725670397281646728515625;-2.456646292673776432735621710889972746372222900390625;0.78551800117602288420215472797281108796596527099609375;-0.7101931466207995757855542251490987837314605712890625;2.164277385897579453200023635872639715671539306640625]
      mask Display: e = 0.06;c1 = [120 150 230]/255;c2 = ([120 150 230]+0)/383;c3 = ([120 150 230]+128)/383;patch([0 1 1 0],[0 0 1 1],c1);patch([0 1 1 1-e 1-e 0+e],[0 0 1 1-e 0+e 0+e],c2);patch([0 0 1 1-e 0+e 0+e],[0 1 1 1-e 1-e 0+e],c3);plot([0 1 1 0 0],[0 0 1 1 0]);disp('Weights');
  "IW{1,1}(57,:)'" : Constant  Value=[-0.7437808595511585796344888876774348318576812744140625;-0.59334758859275760212170780505402944982051849365234375;-2.932153869803707291197270023985765874385833740234375;-0.82056202752617302120796693998272530734539031982421875;-0.161182727550563231755376136788981966674327850341796875;1.25770776305854159460295704775489866733551025390625]
      mask Display: e = 0.06;c1 = [120 150 230]/255;c2 = ([120 150 230]+0)/383;c3 = ([120 150 230]+128)/383;patch([0 1 1 0],[0 0 1 1],c1);patch([0 1 1 1-e 1-e 0+e],[0 0 1 1-e 0+e 0+e],c2);patch([0 0 1 1-e 0+e 0+e],[0 1 1 1-e 1-e 0+e],c3);plot([0 1 1 0 0],[0 0 1 1 0]);disp('Weights');
  "IW{1,1}(58,:)'" : Constant  Value=[1.540287540293778345557029751944355666637420654296875;-1.834311781834541132951699182740412652492523193359375;-0.349397029822331506299093462075688876211643218994140625;0.77546298152566717210021352002513594925403594970703125;-2.1995915770986442794310278259217739105224609375;1.0067006294090805607055472137290053069591522216796875]
      mask Display: e = 0.06;c1 = [120 150 230]/255;c2 = ([120 150 230]+0)/383;c3 = ([120 150 230]+128)/383;patch([0 1 1 0],[0 0 1 1],c1);patch([0 1 1 1-e 1-e 0+e],[0 0 1 1-e 0+e 0+e],c2);patch([0 0 1 1-e 0+e 0+e],[0 1 1 1-e 1-e 0+e],c3);plot([0 1 1 0 0],[0 0 1 1 0]);disp('Weights');
  "IW{1,1}(59,:)'" : Constant  Value=[1.552868240373694419531602761708199977874755859375;0.8140251021753670546132752861012704670429229736328125;1.777790313307401337539204178028739988803863525390625;-1.695296222862948898324475521803833544254302978515625;1.654338500784542365096285720937885344028472900390625;-0.2043946629618224319901997887427569366991519927978515625]
      mask Display: e = 0.06;c1 = [120 150 230]/255;c2 = ([120 150 230]+0)/383;c3 = ([120 150 230]+128)/383;patch([0 1 1 0],[0 0 1 1],c1);patch([0 1 1 1-e 1-e 0+e],[0 0 1 1-e 0+e 0+e],c2);patch([0 0 1 1-e 0+e 0+e],[0 1 1 1-e 1-e 0+e],c3);plot([0 1 1 0 0],[0 0 1 1 0]);disp('Weights');
  "IW{1,1}(6,:)'" : Constant  Value=[-0.85344430298113760358091894886456429958343505859375;1.0621476123359057108785918899229727685451507568359375;1.6940255900231164787328452803194522857666015625;1.6380949105742477200919893220998346805572509765625;-1.91069980432592334551600288250483572483062744140625;0.9956494545299623410983258509077131748199462890625]
      mask Display: e = 0.06;c1 = [120 150 230]/255;c2 = ([120 150 230]+0)/383;c3 = ([120 150 230]+128)/383;patch([0 1 1 0],[0 0 1 1],c1);patch([0 1 1 1-e 1-e 0+e],[0 0 1 1-e 0+e 0+e],c2);patch([0 0 1 1-e 0+e 0+e],[0 1 1 1-e 1-e 0+e],c3);plot([0 1 1 0 0],[0 0 1 1 0]);disp('Weights');
  "IW{1,1}(60,:)'" : Constant  Value=[0.0553679794623206655845848445096635259687900543212890625;1.764112636302499037554980532149784266948699951171875;-1.020500984771047559007683958043344318866729736328125;-1.1473985683300929050432159783667884767055511474609375;2.077832911371721547055813061888329684734344482421875;1.5440680025381496864866903706570155918598175048828125]
      mask Display: e = 0.06;c1 = [120 150 230]/255;c2 = ([120 150 230]+0)/383;c3 = ([120 150 230]+128)/383;patch([0 1 1 0],[0 0 1 1],c1);patch([0 1 1 1-e 1-e 0+e],[0 0 1 1-e 0+e 0+e],c2);patch([0 0 1 1-e 0+e 0+e],[0 1 1 1-e 1-e 0+e],c3);plot([0 1 1 0 0],[0 0 1 1 0]);disp('Weights');
  "IW{1,1}(61,:)'" : Constant  Value=[-2.82528355825135069068210214027203619480133056640625;1.547201964443074562183255693526007235050201416015625;-0.440517759939741182506622863002121448516845703125;0.894107850859394037712490899139083921909332275390625;0.9499629504107065525175812581437639892101287841796875;-0.3592749165716286885441377307870425283908843994140625]
      mask Display: e = 0.06;c1 = [120 150 230]/255;c2 = ([120 150 230]+0)/383;c3 = ([120 150 230]+128)/383;patch([0 1 1 0],[0 0 1 1],c1);patch([0 1 1 1-e 1-e 0+e],[0 0 1 1-e 0+e 0+e],c2);patch([0 0 1 1-e 0+e 0+e],[0 1 1 1-e 1-e 0+e],c3);plot([0 1 1 0 0],[0 0 1 1 0]);disp('Weights');
  "IW{1,1}(62,:)'" : Constant  Value=[-1.372834781478604160298573333420790731906890869140625;-1.18660783004977421484227306791581213474273681640625;-1.533301747370785061974629570613615214824676513671875;1.48866928018520638943300582468509674072265625;1.5072327728224623744068821906694211065769195556640625;1.3401812179252432510878634275286458432674407958984375]
      mask Display: e = 0.06;c1 = [120 150 230]/255;c2 = ([120 150 230]+0)/383;c3 = ([120 150 230]+128)/383;patch([0 1 1 0],[0 0 1 1],c1);patch([0 1 1 1-e 1-e 0+e],[0 0 1 1-e 0+e 0+e],c2);patch([0 0 1 1-e 0+e 0+e],[0 1 1 1-e 1-e 0+e],c3);plot([0 1 1 0 0],[0 0 1 1 0]);disp('Weights');
  "IW{1,1}(63,:)'" : Constant  Value=[1.2701960424788982795263336811331100761890411376953125;-1.3934156868416665009391408602823503315448760986328125;0.889043933303055755601462806225754320621490478515625;-0.1437204150621807230425730494971503503620624542236328125;-2.80968847647668962252964774961583316326141357421875;0.15145508278339792074262959431507624685764312744140625]
      mask Display: e = 0.06;c1 = [120 150 230]/255;c2 = ([120 150 230]+0)/383;c3 = ([120 150 230]+128)/383;patch([0 1 1 0],[0 0 1 1],c1);patch([0 1 1 1-e 1-e 0+e],[0 0 1 1-e 0+e 0+e],c2);patch([0 0 1 1-e 0+e 0+e],[0 1 1 1-e 1-e 0+e],c3);plot([0 1 1 0 0],[0 0 1 1 0]);disp('Weights');
  "IW{1,1}(64,:)'" : Constant  Value=[1.490527369553110492716996304807253181934356689453125;2.36517948192920801631089489092119038105010986328125;0.44061319796056264141981273496639914810657501220703125;-1.630762413845626479513839512947015464305877685546875;0.0876751665492388199130147086179931648075580596923828125;-0.56985784087017077315096003076178021728992462158203125]
